simulink model "Lcontainer_simNN"  (R2018b)
settings: Solver=FixedStepAuto  StartTime=0.0  StopTime=50  FixedStep=0.1  RelTol=1e-3
libraries: neural x548, simulink x2
(part 10 of 26)

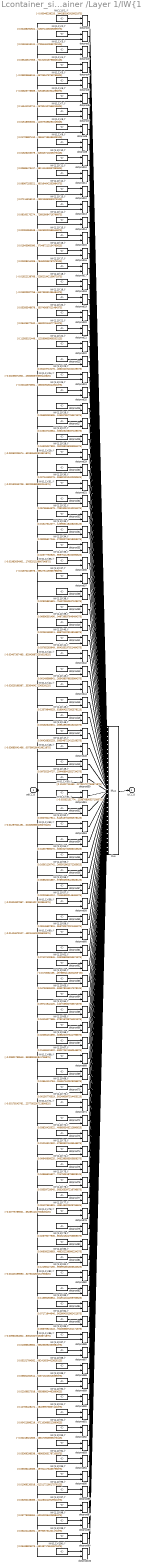
== system Lcontainer_simNN/Lcontainer Plant/NN Plant2 LContainer /Layer 1/IW{1,1} ==
  "pd{1,1}" : Inport  PortDimensions=10
      mask Display: e = 0.06;c1 = [120 230 180]/255;c2 = ([120 230 180]+0)/(256+128);c3 = ([120 230 180]+128)/(256+128);patch([0 1 1 0],[0 0 1 1],c1);patch([0 1 1 1-e 1-e 0+e],[0 0 1 1-e 0+e 0+e],c2);patch([0 0 1 1-e 0+e 0+e],[0 1 1 1-e 1-e 0+e],c3);plot([0 1 1 0 0],[0 0 1 1 0]);
  "IW{1,1}(1,:)'" : Constant  Value=[-0.0094623922020518891340401523848413489758968353271484375;-0.09558953457089498784160497280026902444660663604736328125;0.26068741035971088049194577251910232007503509521484375;-0.0982085917647781136974316495980019681155681610107421875;0.0376402374620294077889326445074402727186679840087890625;0.130169172499156327038605240886681713163852691650390625;0.09123082026825020396376686449002590961754322052001953125;0.08727806527434033012635694603886804543435573577880859375;0.06335140080853875199640157234171056188642978668212890625;-0.019497242791725710731043363921344280242919921875]
      mask Display: e = 0.06;c1 = [120 150 230]/255;c2 = ([120 150 230]+0)/383;c3 = ([120 150 230]+128)/383;patch([0 1 1 0],[0 0 1 1],c1);patch([0 1 1 1-e 1-e 0+e],[0 0 1 1-e 0+e 0+e],c2);patch([0 0 1 1-e 0+e 0+e],[0 1 1 1-e 1-e 0+e],c3);plot([0 1 1 0 0],[0 0 1 1 0]);disp('Weights');
  "IW{1,1}(10,:)'" : Constant  Value=[0.01626203379415903926830111458912142552435398101806640625;-0.0116878579195638099275100785234826616942882537841796875;0.1330582734436684677614692873248714022338390350341796875;0.0022158363261503325435108902041747569455765187740325927734375;-0.054351051398197784692012390905802021734416484832763671875;-0.132257520166433051311827284735045395791530609130859375;0.06380697006039735830196235610856092534959316253662109375;0.249931899969640769487710940666147507727146148681640625;0.1755681253698809507479694502762868069112300872802734375;-0.00686988456380069507922758731410795007832348346710205078125]
      mask Display: e = 0.06;c1 = [120 150 230]/255;c2 = ([120 150 230]+0)/383;c3 = ([120 150 230]+128)/383;patch([0 1 1 0],[0 0 1 1],c1);patch([0 1 1 1-e 1-e 0+e],[0 0 1 1-e 0+e 0+e],c2);patch([0 0 1 1-e 0+e 0+e],[0 1 1 1-e 1-e 0+e],c3);plot([0 1 1 0 0],[0 0 1 1 0]);disp('Weights');
  "IW{1,1}(100,:)'" : Constant  Value=[0.05438825373927226591863615112742991186678409576416015625;-0.061530743551016668646536089681831072084605693817138671875;0.048468771448505997001543477153973071835935115814208984375;-0.01930008978486430493148873210884630680084228515625;-0.053213138463751592788231192798775737173855304718017578125;-0.1481686150629234755005114720916026271879673004150390625;-0.021741347273508182524892617948353290557861328125;0.059229112139614438492518644352458068169653415679931640625;-0.0278726089912357984090807150323598762042820453643798828125;-0.000331265188881957567228198069386735369334928691387176513671875]
      mask Display: e = 0.06;c1 = [120 150 230]/255;c2 = ([120 150 230]+0)/383;c3 = ([120 150 230]+128)/383;patch([0 1 1 0],[0 0 1 1],c1);patch([0 1 1 1-e 1-e 0+e],[0 0 1 1-e 0+e 0+e],c2);patch([0 0 1 1-e 0+e 0+e],[0 1 1 1-e 1-e 0+e],c3);plot([0 1 1 0 0],[0 0 1 1 0]);disp('Weights');
  "IW{1,1}(11,:)'" : Constant  Value=[0.00685473417855186374636478063848699093796312808990478515625;-0.07957314826937157692388069563094177283346652984619140625;0.0831181659954757512398515473250881768763065338134765625;-0.0018459122357845875010695646523117829929105937480926513671875;0.1496921802543421387010624812319292686879634857177734375;0.56792634713675183011361013996065594255924224853515625;0.044275812285080873298426240580738522112369537353515625;0.07070165839502252913550961466171429492533206939697265625;-0.1068912356905150906616341899280087091028690338134765625;0.0091264008795984043198590285328464233316481113433837890625]
      mask Display: e = 0.06;c1 = [120 150 230]/255;c2 = ([120 150 230]+0)/383;c3 = ([120 150 230]+128)/383;patch([0 1 1 0],[0 0 1 1],c1);patch([0 1 1 1-e 1-e 0+e],[0 0 1 1-e 0+e 0+e],c2);patch([0 0 1 1-e 0+e 0+e],[0 1 1 1-e 1-e 0+e],c3);plot([0 1 1 0 0],[0 0 1 1 0]);disp('Weights');
  "IW{1,1}(12,:)'" : Constant  Value=[0.089872555212271276747770798465353436768054962158203125;0.0085118080986059420356415472497246810235083103179931640625;-0.184376627901358058903014125462505035102367401123046875;0.0355803687804530088811816312954761087894439697265625;-0.005487872883921422577369053641405116650275886058807373046875;0.005156923061268266390844150492966946330852806568145751953125;0.11555051477834497875019081902792095206677913665771484375;-0.1686685266223485746284183051102445460855960845947265625;0.085807423146687877846261471859179437160491943359375;0.00411842000985169175153455256577217369340360164642333984375]
      mask Display: e = 0.06;c1 = [120 150 230]/255;c2 = ([120 150 230]+0)/383;c3 = ([120 150 230]+128)/383;patch([0 1 1 0],[0 0 1 1],c1);patch([0 1 1 1-e 1-e 0+e],[0 0 1 1-e 0+e 0+e],c2);patch([0 0 1 1-e 0+e 0+e],[0 1 1 1-e 1-e 0+e],c3);plot([0 1 1 0 0],[0 0 1 1 0]);disp('Weights');
  "IW{1,1}(13,:)'" : Constant  Value=[0.07114816112372672474162271782915922813117504119873046875;-0.032060096051675888995102781109380885027348995208740234375;0.0693593021014935195989181693221325986087322235107421875;0.034399420874747461962517292022312176413834095001220703125;0.02279928598992718435933824139283387921750545501708984375;-0.1450550631977100268787950199111946858465671539306640625;-0.08420904186461160290111394033374381251633167266845703125;0.25200435694978751133277228291262872517108917236328125;-0.060202799283688344933462843755478388629853725433349609375;0.032340333264820504688419333660931442864239215850830078125]
      mask Display: e = 0.06;c1 = [120 150 230]/255;c2 = ([120 150 230]+0)/383;c3 = ([120 150 230]+128)/383;patch([0 1 1 0],[0 0 1 1],c1);patch([0 1 1 1-e 1-e 0+e],[0 0 1 1-e 0+e 0+e],c2);patch([0 0 1 1-e 0+e 0+e],[0 1 1 1-e 1-e 0+e],c3);plot([0 1 1 0 0],[0 0 1 1 0]);disp('Weights');
  "IW{1,1}(14,:)'" : Constant  Value=[0.0816017027410976536483389054410508833825588226318359375;-0.0137702046599115536518187496994869434274733066558837890625;0.061825816425708612911193995387293398380279541015625;0.0182137031645154788550566848925882368348538875579833984375;0.016677444090910188700949134954498731531202793121337890625;-0.039017819642140079416936515599445556290447711944580078125;-0.0167140048186341406977195589433904387988150119781494140625;0.04790839033382394973603624066527117975056171417236328125;-0.08777787377106559263406637683146982453763484954833984375;0.01308305917827646928930374059518726426176726818084716796875]
      mask Display: e = 0.06;c1 = [120 150 230]/255;c2 = ([120 150 230]+0)/383;c3 = ([120 150 230]+128)/383;patch([0 1 1 0],[0 0 1 1],c1);patch([0 1 1 1-e 1-e 0+e],[0 0 1 1-e 0+e 0+e],c2);patch([0 0 1 1-e 0+e 0+e],[0 1 1 1-e 1-e 0+e],c3);plot([0 1 1 0 0],[0 0 1 1 0]);disp('Weights');
  "IW{1,1}(15,:)'" : Constant  Value=[0.0209195394819808623554369120256524183787405490875244140625;-0.009076813538002957704176054676281637512147426605224609375;0.1191679137212347805441226000766619108617305755615234375;0.002321578223835426245391655442062983638606965541839599609375;0.0685148415021334944441377956536598503589630126953125;-0.00157011605704497647119366465773282470763660967350006103515625;0.028108168660927877746669167891013785265386104583740234375;0.09391932602724477330280450360078248195350170135498046875;0.0284578772298975553323163723007382941432297229766845703125;0.005212281091639135548188033197902768733911216259002685546875]
      mask Display: e = 0.06;c1 = [120 150 230]/255;c2 = ([120 150 230]+0)/383;c3 = ([120 150 230]+128)/383;patch([0 1 1 0],[0 0 1 1],c1);patch([0 1 1 1-e 1-e 0+e],[0 0 1 1-e 0+e 0+e],c2);patch([0 0 1 1-e 0+e 0+e],[0 1 1 1-e 1-e 0+e],c3);plot([0 1 1 0 0],[0 0 1 1 0]);disp('Weights');
  "IW{1,1}(16,:)'" : Constant  Value=[0.0184396009007578264016213864806559286080300807952880859375;0.08622273237960843828009416256463737227022647857666015625;0.258984762037696547576359762388165108859539031982421875;0.007701939757252318670410762280198468943126499652862548828125;0.062159638552036954040058702730675577186048030853271484375;-0.11836257965172251871432962389008025638759136199951171875;0.0150200818445607904572103308282748912461102008819580078125;0.1617989899896752070684868840544368140399456024169921875;-0.0188621771444243309379107387258045491762459278106689453125;0.02152205623300353087845593336169258691370487213134765625]
      mask Display: e = 0.06;c1 = [120 150 230]/255;c2 = ([120 150 230]+0)/383;c3 = ([120 150 230]+128)/383;patch([0 1 1 0],[0 0 1 1],c1);patch([0 1 1 1-e 1-e 0+e],[0 0 1 1-e 0+e 0+e],c2);patch([0 0 1 1-e 0+e 0+e],[0 1 1 1-e 1-e 0+e],c3);plot([0 1 1 0 0],[0 0 1 1 0]);disp('Weights');
  "IW{1,1}(17,:)'" : Constant  Value=[0.0230831400684185332472520002511373604647815227508544921875;0.0667508846304031011609225743086426518857479095458984375;0.05900184207744356423841480818737181834876537322998046875;0.0167153228695464568798190185816565644927322864532470703125;-0.000672966141541886928890969787886433550738729536533355712890625;0.1782018798922027913445020885774283669888973236083984375;0.07145595567735839315215429223826504312455654144287109375;0.04002558594403750336088165795445092953741550445556640625;-0.1367353179557696252199860964537947438657283782958984375;0.004458470848905435497677718359454956953413784503936767578125]
      mask Display: e = 0.06;c1 = [120 150 230]/255;c2 = ([120 150 230]+0)/383;c3 = ([120 150 230]+128)/383;patch([0 1 1 0],[0 0 1 1],c1);patch([0 1 1 1-e 1-e 0+e],[0 0 1 1-e 0+e 0+e],c2);patch([0 0 1 1-e 0+e 0+e],[0 1 1 1-e 1-e 0+e],c3);plot([0 1 1 0 0],[0 0 1 1 0]);disp('Weights');
  "IW{1,1}(18,:)'" : Constant  Value=[-0.0182213876655290263339992407054523937404155731201171875;-0.000399743420678597030475109885827578182215802371501922607421875;-0.050901316682216070363953264177325763739645481109619140625;0.0250893053095773109484323271090033813379704952239990234375;0.08090673602776325690211223218284430913627147674560546875;0.0938809802481468669288489081736770458519458770751953125;0.0198702950067176260795509534773373161442577838897705078125;-0.057703964383789975445271380749545642174780368804931640625;-0.04276041067470219558810384796743164770305156707763671875;0.01306358593354533907671122250349071691744029521942138671875]
      mask Display: e = 0.06;c1 = [120 150 230]/255;c2 = ([120 150 230]+0)/383;c3 = ([120 150 230]+128)/383;patch([0 1 1 0],[0 0 1 1],c1);patch([0 1 1 1-e 1-e 0+e],[0 0 1 1-e 0+e 0+e],c2);patch([0 0 1 1-e 0+e 0+e],[0 1 1 1-e 1-e 0+e],c3);plot([0 1 1 0 0],[0 0 1 1 0]);disp('Weights');
  "IW{1,1}(19,:)'" : Constant  Value=[-0.018209377569535119267829514910772559233009815216064453125;-0.016649902739864948231218733099012752063572406768798828125;-0.004527751093878955822302767586506888619624078273773193359375;-0.0068852252691341438162186960880717379041016101837158203125;0.02209772471243469371682266455536591820418834686279296875;0.046415344483233873795757773450532113201916217803955078125;-0.004664568795302062066687742714066189364530146121978759765625;-0.01713973095097658105867566291635739617049694061279296875;-0.01135203955323040893310437837726567522622644901275634765625;-0.008753261637478436385517710505155264399945735931396484375]
      mask Display: e = 0.06;c1 = [120 150 230]/255;c2 = ([120 150 230]+0)/383;c3 = ([120 150 230]+128)/383;patch([0 1 1 0],[0 0 1 1],c1);patch([0 1 1 1-e 1-e 0+e],[0 0 1 1-e 0+e 0+e],c2);patch([0 0 1 1-e 0+e 0+e],[0 1 1 1-e 1-e 0+e],c3);plot([0 1 1 0 0],[0 0 1 1 0]);disp('Weights');
  "IW{1,1}(2,:)'" : Constant  Value=[0.004882929243012936425250014593757441616617143154144287109375;-0.057596398999574770216636210307115106843411922454833984375;-0.044082564852459558968345021412460482679307460784912109375;-0.01406400921559781795611154819880539434961974620819091796875;-0.0207834799436826568597158626516829826869070529937744140625;-0.12500641299832937480829286869266070425510406494140625;0.010192874151138286986650882681715302169322967529296875;0.08502904507598389727274224014763603918254375457763671875;0.141777425947241242365493008037446998059749603271484375;0.002150746476123398774615846917868111631833016872406005859375]
      mask Display: e = 0.06;c1 = [120 150 230]/255;c2 = ([120 150 230]+0)/383;c3 = ([120 150 230]+128)/383;patch([0 1 1 0],[0 0 1 1],c1);patch([0 1 1 1-e 1-e 0+e],[0 0 1 1-e 0+e 0+e],c2);patch([0 0 1 1-e 0+e 0+e],[0 1 1 1-e 1-e 0+e],c3);plot([0 1 1 0 0],[0 0 1 1 0]);disp('Weights');
  "IW{1,1}(20,:)'" : Constant  Value=[0.053935486796124150477016456761703011579811573028564453125;-0.0031300549363098115369929974605156530742533504962921142578125;0.09777932299305640284625695812792400829493999481201171875;-0.0341856829207596302211413785698823630809783935546875;0.1637615555876408279800671152770519256591796875;0.55379762131474119524199295483413152396678924560546875;0.049984170569442522291669916967293829657137393951416015625;-0.239524968831588969120360843589878641068935394287109375;0.1618070812272489888972160088087548501789569854736328125;0.027466021220655834067514433627366088330745697021484375]
      mask Display: e = 0.06;c1 = [120 150 230]/255;c2 = ([120 150 230]+0)/383;c3 = ([120 150 230]+128)/383;patch([0 1 1 0],[0 0 1 1],c1);patch([0 1 1 1-e 1-e 0+e],[0 0 1 1-e 0+e 0+e],c2);patch([0 0 1 1-e 0+e 0+e],[0 1 1 1-e 1-e 0+e],c3);plot([0 1 1 0 0],[0 0 1 1 0]);disp('Weights');
  "IW{1,1}(21,:)'" : Constant  Value=[0.054256779428249753138846500633007963187992572784423828125;-0.11238736437717598837249255439019179902970790863037109375;-0.1293053208545835996989836758075398392975330352783203125;0.0220913833444768455127604767085358616895973682403564453125;-0.03223635894362240905675065505420207045972347259521484375;0.10098705478395973711425170904476544819772243499755859375;-0.019627013149193052454766217351789237000048160552978515625;0.061199006731056944385915841166934114880859851837158203125;0.084865917404867874385132608949788846075534820556640625;0.04309910366681900251162318227216019295156002044677734375]
      mask Display: e = 0.06;c1 = [120 150 230]/255;c2 = ([120 150 230]+0)/383;c3 = ([120 150 230]+128)/383;patch([0 1 1 0],[0 0 1 1],c1);patch([0 1 1 1-e 1-e 0+e],[0 0 1 1-e 0+e 0+e],c2);patch([0 0 1 1-e 0+e 0+e],[0 1 1 1-e 1-e 0+e],c3);plot([0 1 1 0 0],[0 0 1 1 0]);disp('Weights');
  "IW{1,1}(22,:)'" : Constant  Value=[0.1158315144990087475207474199123680591583251953125;-0.1634728196516810616589765459139016456902027130126953125;0.035020493849886764892165302853754837997257709503173828125;0.0111778835228135246804281877075482043437659740447998046875;-0.0561490815014391575488161834073252975940704345703125;-0.2146205341687602297096049142055562697350978851318359375;0.11055470925725384423454755733473575673997402191162109375;0.0154180878450160437076466024564069812186062335968017578125;0.066143219849594092618616514300811104476451873779296875;0.033149436754358004020293293478971463628113269805908203125]
      mask Display: e = 0.06;c1 = [120 150 230]/255;c2 = ([120 150 230]+0)/383;c3 = ([120 150 230]+128)/383;patch([0 1 1 0],[0 0 1 1],c1);patch([0 1 1 1-e 1-e 0+e],[0 0 1 1-e 0+e 0+e],c2);patch([0 0 1 1-e 0+e 0+e],[0 1 1 1-e 1-e 0+e],c3);plot([0 1 1 0 0],[0 0 1 1 0]);disp('Weights');
  "IW{1,1}(23,:)'" : Constant  Value=[0.00419713176387549909140961545972459134645760059356689453125;0.1170293572207423693498640204779803752899169921875;0.05992652827845613983104300359627814032137393951416015625;0.0027034221247037859559014805199694819748401641845703125;-0.0184799404250086708734190921177287236787378787994384765625;0.1485927881894391067163496700231917202472686767578125;-0.053373316924542467398762113361954106949269771575927734375;-0.041164967862770511508596626981670851819217205047607421875;0.0661805237237923782434023678433732129633426666259765625;0.00348532813765325098775971213171942508779466152191162109375]
      mask Display: e = 0.06;c1 = [120 150 230]/255;c2 = ([120 150 230]+0)/383;c3 = ([120 150 230]+128)/383;patch([0 1 1 0],[0 0 1 1],c1);patch([0 1 1 1-e 1-e 0+e],[0 0 1 1-e 0+e 0+e],c2);patch([0 0 1 1-e 0+e 0+e],[0 1 1 1-e 1-e 0+e],c3);plot([0 1 1 0 0],[0 0 1 1 0]);disp('Weights');
  "IW{1,1}(24,:)'" : Constant  Value=[-0.0023667490167734671867305618064847294590435922145843505859375;-0.0026621574457762827055351539939920257893390953540802001953125;0.098039684675983007622335207997821271419525146484375;0.0219371829502120647970020428374482435174286365509033203125;-0.02163029214711008341165410229223198257386684417724609375;0.1095352711170798354345379266305826604366302490234375;-0.01500366036165250681333471760581232956610620021820068359375;0.04497043112273464704475856024146196432411670684814453125;-0.025171986185772356192646981298821629025042057037353515625;0.01015432471195599518909435943214703002013266086578369140625]
      mask Display: e = 0.06;c1 = [120 150 230]/255;c2 = ([120 150 230]+0)/383;c3 = ([120 150 230]+128)/383;patch([0 1 1 0],[0 0 1 1],c1);patch([0 1 1 1-e 1-e 0+e],[0 0 1 1-e 0+e 0+e],c2);patch([0 0 1 1-e 0+e 0+e],[0 1 1 1-e 1-e 0+e],c3);plot([0 1 1 0 0],[0 0 1 1 0]);disp('Weights');
  "IW{1,1}(25,:)'" : Constant  Value=[-0.000428708940112308288690468049964010788244195282459259033203125;9.1544086241367931926216083837744008633308112621307373046875e-05;-0.0004300533793372667413883181364298025073367170989513397216796875;6.48029488285427335281241312259226106107234954833984375e-05;-0.00129145474964229727866948937986535383970476686954498291015625;-0.0020837039570330271633091800964621143066324293613433837890625;-0.0004094497946522885679400405312122757095494307577610015869140625;0.0001162733233937415983950958153769761338480748236179351806640625;-0.00016801208466965373796754568136435636915848590433597564697265625;-0.0002100271527808877133729204000900381288374774158000946044921875]
      mask Display: e = 0.06;c1 = [120 150 230]/255;c2 = ([120 150 230]+0)/383;c3 = ([120 150 230]+128)/383;patch([0 1 1 0],[0 0 1 1],c1);patch([0 1 1 1-e 1-e 0+e],[0 0 1 1-e 0+e 0+e],c2);patch([0 0 1 1-e 0+e 0+e],[0 1 1 1-e 1-e 0+e],c3);plot([0 1 1 0 0],[0 0 1 1 0]);disp('Weights');
  "IW{1,1}(26,:)'" : Constant  Value=[0.055892806950742328353509691396538983099162578582763671875;-0.1284268204621448195013044824008829891681671142578125;-0.0635938515163453066403320690369582735002040863037109375;0.0278544960430266476392180408083731890656054019927978515625;0.0018930102148548813741080198980171189759857952594757080078125;-0.090385076943400533000527730109752155840396881103515625;0.132461038461452684789065870063495822250843048095703125;0.13139818141287362696090212921262718737125396728515625;0.1367989270820009484186385861903545446693897247314453125;-0.0002401367004118174180819778040785195116768591105937957763671875]
      mask Display: e = 0.06;c1 = [120 150 230]/255;c2 = ([120 150 230]+0)/383;c3 = ([120 150 230]+128)/383;patch([0 1 1 0],[0 0 1 1],c1);patch([0 1 1 1-e 1-e 0+e],[0 0 1 1-e 0+e 0+e],c2);patch([0 0 1 1-e 0+e 0+e],[0 1 1 1-e 1-e 0+e],c3);plot([0 1 1 0 0],[0 0 1 1 0]);disp('Weights');
  "IW{1,1}(27,:)'" : Constant  Value=[0.1061671838416390067916239559053792618215084075927734375;0.01455106568329974682518557216326371417380869388580322265625;0.2194665097169405110211215514937066473066806793212890625;0.01436225965540223643845951784214776125736534595489501953125;-0.0997290353010053809423851589599507860839366912841796875;-0.51024718783592548643213149262010119855403900146484375;-7.5215616431395691744883624796358390085515566170215606689453125e-05;0.046546095145313791385799362387842847965657711029052734375;-0.054755540426459102520961863547199754975736141204833984375;-0.01035067696942139868487853249234831309877336025238037109375]
      mask Display: e = 0.06;c1 = [120 150 230]/255;c2 = ([120 150 230]+0)/383;c3 = ([120 150 230]+128)/383;patch([0 1 1 0],[0 0 1 1],c1);patch([0 1 1 1-e 1-e 0+e],[0 0 1 1-e 0+e 0+e],c2);patch([0 0 1 1-e 0+e 0+e],[0 1 1 1-e 1-e 0+e],c3);plot([0 1 1 0 0],[0 0 1 1 0]);disp('Weights');
  "IW{1,1}(28,:)'" : Constant  Value=[0.043250379936406797842796123632069793529808521270751953125;0.049753204596124860070727180527683231048285961151123046875;-0.1329378169960137856531190436726319603621959686279296875;0.01885286933153483557301655082483193837106227874755859375;0.046117914719532533684986930211380240507423877716064453125;0.35414050109305106328605461385450325906276702880859375;-0.033653993165451250024755580625424045138061046600341796875;-0.003085228111936642002299802101106251939199864864349365234375;-0.07851150253082912755520084147065063007175922393798828125;0.036814308916874725896573039563008933328092098236083984375]
      mask Display: e = 0.06;c1 = [120 150 230]/255;c2 = ([120 150 230]+0)/383;c3 = ([120 150 230]+128)/383;patch([0 1 1 0],[0 0 1 1],c1);patch([0 1 1 1-e 1-e 0+e],[0 0 1 1-e 0+e 0+e],c2);patch([0 0 1 1-e 0+e 0+e],[0 1 1 1-e 1-e 0+e],c3);plot([0 1 1 0 0],[0 0 1 1 0]);disp('Weights');
  "IW{1,1}(29,:)'" : Constant  Value=[-0.030620255742750242256011716790453647263348102569580078125;-0.060072751731736630242952656999477767385542392730712890625;0.035252039674856010254000437953436630778014659881591796875;-0.00919170816308433925867493741179714561440050601959228515625;0.023535161861715871156608415049049654044210910797119140625;0.2258211689467672644848761365210521034896373748779296875;-0.00230639337737633016989224898907195893116295337677001953125;0.007157763388058989602324988510417824727483093738555908203125;-0.1325624286244390936939652192450012080371379852294921875;-0.00019654571167457865303596076245185031439177691936492919921875]
      mask Display: e = 0.06;c1 = [120 150 230]/255;c2 = ([120 150 230]+0)/383;c3 = ([120 150 230]+128)/383;patch([0 1 1 0],[0 0 1 1],c1);patch([0 1 1 1-e 1-e 0+e],[0 0 1 1-e 0+e 0+e],c2);patch([0 0 1 1-e 0+e 0+e],[0 1 1 1-e 1-e 0+e],c3);plot([0 1 1 0 0],[0 0 1 1 0]);disp('Weights');
  "IW{1,1}(3,:)'" : Constant  Value=[0.01504613241257331084088644246321564423851668834686279296875;-0.018507599401025205676507567886801552958786487579345703125;0.0418247693695602273944444959852262400090694427490234375;-0.09051438570647639403343731601125909946858882904052734375;-0.0171372621545999026526629904765286482870578765869140625;-0.170833727731954432282890365968341939151287078857421875;-0.0035696038583175608745190476867037432384677231311798095703125;-0.034239869832726803344780108773193205706775188446044921875;0.0251699400853839481972951119814752019010484218597412109375;-0.000573952465504741493607099300788831897079944610595703125]
      mask Display: e = 0.06;c1 = [120 150 230]/255;c2 = ([120 150 230]+0)/383;c3 = ([120 150 230]+128)/383;patch([0 1 1 0],[0 0 1 1],c1);patch([0 1 1 1-e 1-e 0+e],[0 0 1 1-e 0+e 0+e],c2);patch([0 0 1 1-e 0+e 0+e],[0 1 1 1-e 1-e 0+e],c3);plot([0 1 1 0 0],[0 0 1 1 0]);disp('Weights');
  "IW{1,1}(30,:)'" : Constant  Value=[0.027341892766545104753728168134330189786851406097412109375;0.1252022346316188639026023565747891552746295928955078125;-0.0110998452900594561654212810708486358635127544403076171875;0.049645084866596599082466667596236220560967922210693359375;-0.04948149832591917929303093615089892409741878509521484375;-0.059672753066025006896122562238815589807927608489990234375;0.021246913175135127838100146391298039816319942474365234375;0.10083037720781040658124538822448812425136566162109375;0.0601722007103199507671575929634855128824710845947265625;0.005628721429224396201329572164695491665042936801910400390625]
      mask Display: e = 0.06;c1 = [120 150 230]/255;c2 = ([120 150 230]+0)/383;c3 = ([120 150 230]+128)/383;patch([0 1 1 0],[0 0 1 1],c1);patch([0 1 1 1-e 1-e 0+e],[0 0 1 1-e 0+e 0+e],c2);patch([0 0 1 1-e 0+e 0+e],[0 1 1 1-e 1-e 0+e],c3);plot([0 1 1 0 0],[0 0 1 1 0]);disp('Weights');
  "IW{1,1}(31,:)'" : Constant  Value=[-0.001300457083481666546720401100856179255060851573944091796875;0.0029817332399571555741346617907083782483823597431182861328125;-0.0035784949147766999082154182332260461407713592052459716796875;0.004177790401596108600668078025819340837188065052032470703125;-0.01019553427399688162735547081183540285564959049224853515625;-0.0160996964297110585484507083720018272288143634796142578125;-0.002441254860139726277912242125012198812328279018402099609375;0.0031805179703750029000797194811411827686242759227752685546875;-0.000631347408235451829604245599369960473268292844295501708984375;-0.000638603839496102907401231529860297086997888982295989990234375]
      mask Display: e = 0.06;c1 = [120 150 230]/255;c2 = ([120 150 230]+0)/383;c3 = ([120 150 230]+128)/383;patch([0 1 1 0],[0 0 1 1],c1);patch([0 1 1 1-e 1-e 0+e],[0 0 1 1-e 0+e 0+e],c2);patch([0 0 1 1-e 0+e 0+e],[0 1 1 1-e 1-e 0+e],c3);plot([0 1 1 0 0],[0 0 1 1 0]);disp('Weights');
  "IW{1,1}(32,:)'" : Constant  Value=[0.057655645798538823765255756370606832206249237060546875;0.0175213535064214949443783808646912802942097187042236328125;0.167545314656773414174750769234378822147846221923828125;0.01435359908537950542062322512038008426316082477569580078125;-0.0424012483635934633863229237249470315873622894287109375;-0.1755816998638709824920312030371860601007938385009765625;-0.026032023806178118674470312043922604061663150787353515625;0.1070502049234766384078199052964919246733188629150390625;-0.04798256895018682133269294354249723255634307861328125;0.023793277194497496063174679648000164888799190521240234375]
      mask Display: e = 0.06;c1 = [120 150 230]/255;c2 = ([120 150 230]+0)/383;c3 = ([120 150 230]+128)/383;patch([0 1 1 0],[0 0 1 1],c1);patch([0 1 1 1-e 1-e 0+e],[0 0 1 1-e 0+e 0+e],c2);patch([0 0 1 1-e 0+e 0+e],[0 1 1 1-e 1-e 0+e],c3);plot([0 1 1 0 0],[0 0 1 1 0]);disp('Weights');
  "IW{1,1}(33,:)'" : Constant  Value=[0.0154751207722963191049103670593467541038990020751953125;-0.06508292427735633267626980114073376171290874481201171875;0.003597379266779768790252003185514695360325276851654052734375;-0.01217999549635321275553589970286338939331471920013427734375;-0.024807022455973541663620807184997829608619213104248046875;0.245955434496933078580838127891183830797672271728515625;0.054715556931545165919583695313122007064521312713623046875;0.00124258971353589388851579311534578664577566087245941162109375;0.044862425392990117056779553195156040601432323455810546875;0.0021306295208748525678299490238032376510091125965118408203125]
      mask Display: e = 0.06;c1 = [120 150 230]/255;c2 = ([120 150 230]+0)/383;c3 = ([120 150 230]+128)/383;patch([0 1 1 0],[0 0 1 1],c1);patch([0 1 1 1-e 1-e 0+e],[0 0 1 1-e 0+e 0+e],c2);patch([0 0 1 1-e 0+e 0+e],[0 1 1 1-e 1-e 0+e],c3);plot([0 1 1 0 0],[0 0 1 1 0]);disp('Weights');
  "IW{1,1}(34,:)'" : Constant  Value=[0.0829561724641332265406390433781780302524566650390625;-0.08643372278495968508149616127411718480288982391357421875;0.02650072339475682825504776474190293811261653900146484375;-0.010102262395204252010127987659870996139943599700927734375;-0.0170359998743756478611910409881602390669286251068115234375;-0.2137723706639365894854876160025014542043209075927734375;0.1662215532799683204157048521665274165570735931396484375;0.1793015865651973184125012039658031426370143890380859375;0.044423895055723854052853738494377466849982738494873046875;0.006377591494637540291134936154548995546065270900726318359375]
      mask Display: e = 0.06;c1 = [120 150 230]/255;c2 = ([120 150 230]+0)/383;c3 = ([120 150 230]+128)/383;patch([0 1 1 0],[0 0 1 1],c1);patch([0 1 1 1-e 1-e 0+e],[0 0 1 1-e 0+e 0+e],c2);patch([0 0 1 1-e 0+e 0+e],[0 1 1 1-e 1-e 0+e],c3);plot([0 1 1 0 0],[0 0 1 1 0]);disp('Weights');
  "IW{1,1}(35,:)'" : Constant  Value=[0.0257775092536612245031069079459484783001244068145751953125;0.01013277491170373571793827949250044184736907482147216796875;0.1824594839372037646807456212627585045993328094482421875;-0.037732190422867024903741395291945082135498523712158203125;0.116527238491814066900786883707041852176189422607421875;0.446641372272815695421144255305989645421504974365234375;0.051285192038531483837981994611254776827991008758544921875;-0.049995574103856306458215641441711341030895709991455078125;-0.023550005796922769685242116111112409271299839019775390625;0.03835423208526923810612885290538542903959751129150390625]
      mask Display: e = 0.06;c1 = [120 150 230]/255;c2 = ([120 150 230]+0)/383;c3 = ([120 150 230]+128)/383;patch([0 1 1 0],[0 0 1 1],c1);patch([0 1 1 1-e 1-e 0+e],[0 0 1 1-e 0+e 0+e],c2);patch([0 0 1 1-e 0+e 0+e],[0 1 1 1-e 1-e 0+e],c3);plot([0 1 1 0 0],[0 0 1 1 0]);disp('Weights');
  "IW{1,1}(36,:)'" : Constant  Value=[-0.01983054901434673500393301992517081089317798614501953125;0.018452101329059479584149272568538435734808444976806640625;0.0032003306650281028271354255565483981627039611339569091796875;0.0189674161409785456411380977215230814181268215179443359375;-0.045544104438170647519701361716215615160763263702392578125;0.11854060794901606634699220421680365689098834991455078125;-0.03286269016840230594578287082185852341353893280029296875;0.2297929534733335332763459746274747885763645172119140625;0.2591117873913864055879230363643728196620941162109375;-0.0021468140763482713821719283231459485250525176525115966796875]
      mask Display: e = 0.06;c1 = [120 150 230]/255;c2 = ([120 150 230]+0)/383;c3 = ([120 150 230]+128)/383;patch([0 1 1 0],[0 0 1 1],c1);patch([0 1 1 1-e 1-e 0+e],[0 0 1 1-e 0+e 0+e],c2);patch([0 0 1 1-e 0+e 0+e],[0 1 1 1-e 1-e 0+e],c3);plot([0 1 1 0 0],[0 0 1 1 0]);disp('Weights');
  "IW{1,1}(37,:)'" : Constant  Value=[-0.01870216976054601965007151420650188811123371124267578125;-0.1487696091116151586586369148790254257619380950927734375;-0.042997654762433688835354672619359917007386684417724609375;-0.0157909863387145910085251898635760881006717681884765625;0.060172801600213599027000554997357539832592010498046875;0.295341177415798628036469608559855259954929351806640625;0.04437611723870467372865533661752124316990375518798828125;0.057450552118198931761394732120606931857764720916748046875;0.1758418061116827912915283604888827539980411529541015625;0.01235623289356558955620624118409978109411895275115966796875]
      mask Display: e = 0.06;c1 = [120 150 230]/255;c2 = ([120 150 230]+0)/383;c3 = ([120 150 230]+128)/383;patch([0 1 1 0],[0 0 1 1],c1);patch([0 1 1 1-e 1-e 0+e],[0 0 1 1-e 0+e 0+e],c2);patch([0 0 1 1-e 0+e 0+e],[0 1 1 1-e 1-e 0+e],c3);plot([0 1 1 0 0],[0 0 1 1 0]);disp('Weights');
  "IW{1,1}(38,:)'" : Constant  Value=[0.02925881681080506890868520031290245242416858673095703125;0.091494353634817338072338088750257156789302825927734375;-0.0067900404159471593190655624994178651832044124603271484375;0.006873783434484160952127052013338470715098083019256591796875;0.010202439038604564636170124458658392541110515594482421875;-0.0069640709699677165456233041140876593999564647674560546875;0.04781638241289569435377160289135645143687725067138671875;-0.041503627391795409884434064906599815003573894500732421875;-0.047215748285432075637135795886933919973671436309814453125;-0.000644734460318443516023412254156710332608781754970550537109375]
      mask Display: e = 0.06;c1 = [120 150 230]/255;c2 = ([120 150 230]+0)/383;c3 = ([120 150 230]+128)/383;patch([0 1 1 0],[0 0 1 1],c1);patch([0 1 1 1-e 1-e 0+e],[0 0 1 1-e 0+e 0+e],c2);patch([0 0 1 1-e 0+e 0+e],[0 1 1 1-e 1-e 0+e],c3);plot([0 1 1 0 0],[0 0 1 1 0]);disp('Weights');
  "IW{1,1}(39,:)'" : Constant  Value=[0.06696391490814442015722107726105605252087116241455078125;0.043507059958706455204957563864809344522655010223388671875;0.0022627982478876872661499586314448606572113931179046630859375;0.00592600017327450136195299279506798484362661838531494140625;0.024770048623384478825304455540390335954725742340087890625;-0.2191043250452577861864256192347966134548187255859375;0.024279235658779714512878200594059308059513568878173828125;0.136827226052908812459207865686039440333843231201171875;0.12302496885916480717781951170763932168483734130859375;0.042787993807286893443997399799627601169049739837646484375]
      mask Display: e = 0.06;c1 = [120 150 230]/255;c2 = ([120 150 230]+0)/383;c3 = ([120 150 230]+128)/383;patch([0 1 1 0],[0 0 1 1],c1);patch([0 1 1 1-e 1-e 0+e],[0 0 1 1-e 0+e 0+e],c2);patch([0 0 1 1-e 0+e 0+e],[0 1 1 1-e 1-e 0+e],c3);plot([0 1 1 0 0],[0 0 1 1 0]);disp('Weights');
  "IW{1,1}(4,:)'" : Constant  Value=[0.036406173535373155536465361592490808106958866119384765625;0.0303225872789273688534539274996859603561460971832275390625;0.016992587776736754745510182829093537293374538421630859375;0.0712699496276618382761824932458694092929363250732421875;-0.0922836711084928651427361501191626302897930145263671875;-0.0293263071250228178621366481593213393352925777435302734375;0.003353206534465286332846734040913361241109669208526611328125;0.003514382330419968218648829605399441788904368877410888671875;-0.07268810781557318023704539200480212457478046417236328125;-0.0020694202711757825503824381740969329257495701313018798828125]
      mask Display: e = 0.06;c1 = [120 150 230]/255;c2 = ([120 150 230]+0)/383;c3 = ([120 150 230]+128)/383;patch([0 1 1 0],[0 0 1 1],c1);patch([0 1 1 1-e 1-e 0+e],[0 0 1 1-e 0+e 0+e],c2);patch([0 0 1 1-e 0+e 0+e],[0 1 1 1-e 1-e 0+e],c3);plot([0 1 1 0 0],[0 0 1 1 0]);disp('Weights');
  "IW{1,1}(40,:)'" : Constant  Value=[0.0226246931135768401810448580135926022194325923919677734375;0.0609845520991494083329342856814037077128887176513671875;0.11617872595918903033673785785140353254973888397216796875;-0.0114620108114807418842051589535913080908358097076416015625;0.08985106470019448010599916187857161276042461395263671875;0.423456091179193749862719187149195931851863861083984375;-0.0841011889559413472472471084984135814011096954345703125;-0.032343871456650685747291618099552579224109649658203125;0.0187508808586528304129803501609785598702728748321533203125;0.053166644332708561104805511376980575732886791229248046875]
      mask Display: e = 0.06;c1 = [120 150 230]/255;c2 = ([120 150 230]+0)/383;c3 = ([120 150 230]+128)/383;patch([0 1 1 0],[0 0 1 1],c1);patch([0 1 1 1-e 1-e 0+e],[0 0 1 1-e 0+e 0+e],c2);patch([0 0 1 1-e 0+e 0+e],[0 1 1 1-e 1-e 0+e],c3);plot([0 1 1 0 0],[0 0 1 1 0]);disp('Weights');
  "IW{1,1}(41,:)'" : Constant  Value=[0.037652839492859212222608533693346544168889522552490234375;0.0706526518036562911628806205044384114444255828857421875;0.11989744985270396615550936303407070226967334747314453125;0.00365966674761863085263424721915725967846810817718505859375;0.017277339343304609631246648859814740717411041259765625;0.135125244957386814181887757513322867453098297119140625;0.00192273184513320843057326836600395836285315454006195068359375;-0.03252992580396761590488807769361301325261592864990234375;-0.102432590640903875556233515453641302883625030517578125;0.0065013752071739171201070206507210968993604183197021484375]
      mask Display: e = 0.06;c1 = [120 150 230]/255;c2 = ([120 150 230]+0)/383;c3 = ([120 150 230]+128)/383;patch([0 1 1 0],[0 0 1 1],c1);patch([0 1 1 1-e 1-e 0+e],[0 0 1 1-e 0+e 0+e],c2);patch([0 0 1 1-e 0+e 0+e],[0 1 1 1-e 1-e 0+e],c3);plot([0 1 1 0 0],[0 0 1 1 0]);disp('Weights');
  "IW{1,1}(42,:)'" : Constant  Value=[-0.034073074951517672015466331458810600452125072479248046875;0.0789402390914708818048239891140838153660297393798828125;0.0226947690121968824461529123936998075805604457855224609375;-0.0186643067981428732726723040968863642774522304534912109375;0.0280594575673095876500173773138158139772713184356689453125;0.27117506491122245204650198502349667251110076904296875;-0.054575703267962301368232402865032781846821308135986328125;0.0295706673640438420791465290449195890687406063079833984375;-0.1193862284205201851339239738081232644617557525634765625;-0.00906888053951409624231505546276821405626833438873291015625]
      mask Display: e = 0.06;c1 = [120 150 230]/255;c2 = ([120 150 230]+0)/383;c3 = ([120 150 230]+128)/383;patch([0 1 1 0],[0 0 1 1],c1);patch([0 1 1 1-e 1-e 0+e],[0 0 1 1-e 0+e 0+e],c2);patch([0 0 1 1-e 0+e 0+e],[0 1 1 1-e 1-e 0+e],c3);plot([0 1 1 0 0],[0 0 1 1 0]);disp('Weights');
  "IW{1,1}(43,:)'" : Constant  Value=[0.00149588641771458458369636890239462445606477558612823486328125;0.028824063696041679616399733276921324431896209716796875;0.034845924388722006315166623835466452874243259429931640625;-0.0272887302741802069416809928270595264621078968048095703125;0.05041316221349168014143060645437799394130706787109375;0.09148685717208689116564102050688234157860279083251953125;-0.10707755038642419176397879709838889539241790771484375;0.00887624718988880463677038079595149611122906208038330078125;-0.0960741601912546705488438192332978360354900360107421875;-0.0025010786829252340535134635501890443265438079833984375]
      mask Display: e = 0.06;c1 = [120 150 230]/255;c2 = ([120 150 230]+0)/383;c3 = ([120 150 230]+128)/383;patch([0 1 1 0],[0 0 1 1],c1);patch([0 1 1 1-e 1-e 0+e],[0 0 1 1-e 0+e 0+e],c2);patch([0 0 1 1-e 0+e 0+e],[0 1 1 1-e 1-e 0+e],c3);plot([0 1 1 0 0],[0 0 1 1 0]);disp('Weights');
  "IW{1,1}(44,:)'" : Constant  Value=[-0.0262919838708194873733159369066925137303769588470458984375;-0.09891711576821389517721883066769805736839771270751953125;0.171248082329450823646510571052203886210918426513671875;-0.031560906234920249602282638079486787319183349609375;0.0763710517151593715201585155227803625166416168212890625;0.84927724511108915184109946494572795927524566650390625;0.0881912324052968876753055837980355136096477508544921875;0.1364688751119919885024245331806014291942119598388671875;0.0151534903671480015996397838762277388013899326324462890625;0.00538303845850146740759090135952646960504353046417236328125]
      mask Display: e = 0.06;c1 = [120 150 230]/255;c2 = ([120 150 230]+0)/383;c3 = ([120 150 230]+128)/383;patch([0 1 1 0],[0 0 1 1],c1);patch([0 1 1 1-e 1-e 0+e],[0 0 1 1-e 0+e 0+e],c2);patch([0 0 1 1-e 0+e 0+e],[0 1 1 1-e 1-e 0+e],c3);plot([0 1 1 0 0],[0 0 1 1 0]);disp('Weights');
  "IW{1,1}(45,:)'" : Constant  Value=[0.13379846033323306020434984020539559423923492431640625;0.041478146715528636800929263017678749747574329376220703125;-0.08059196209386564058174684532787068746984004974365234375;0.03778851120177016686962900848811841569840908050537109375;-0.005282945967682390643604950497547179111279547214508056640625;-0.1279698649768603591070359470904804766178131103515625;-0.019188878855175194038107377991764224134385585784912109375;-0.01211062158931112790749562435621555778197944164276123046875;0.09436972662845211079485352456686086952686309814453125;0.03765781897895577323698290683751110918819904327392578125]
      mask Display: e = 0.06;c1 = [120 150 230]/255;c2 = ([120 150 230]+0)/383;c3 = ([120 150 230]+128)/383;patch([0 1 1 0],[0 0 1 1],c1);patch([0 1 1 1-e 1-e 0+e],[0 0 1 1-e 0+e 0+e],c2);patch([0 0 1 1-e 0+e 0+e],[0 1 1 1-e 1-e 0+e],c3);plot([0 1 1 0 0],[0 0 1 1 0]);disp('Weights');
  "IW{1,1}(46,:)'" : Constant  Value=[0.031826406319517393239681979366650921292603015899658203125;0.09134328812660989782568066175372223369777202606201171875;0.1876069824791513074302429231465794146060943603515625;-0.021759602034773894985164588433690369129180908203125;-0.1273349733162982833079013289534486830234527587890625;-0.2930394475669177989374247772502712905406951904296875;0.0190227768760909791978530591904927860014140605926513671875;0.01162750862308703676817334127235881169326603412628173828125;-0.019561777479921334255141829316926305182278156280517578125;0.006964629140588782761633890316943507059477269649505615234375]
      mask Display: e = 0.06;c1 = [120 150 230]/255;c2 = ([120 150 230]+0)/383;c3 = ([120 150 230]+128)/383;patch([0 1 1 0],[0 0 1 1],c1);patch([0 1 1 1-e 1-e 0+e],[0 0 1 1-e 0+e 0+e],c2);patch([0 0 1 1-e 0+e 0+e],[0 1 1 1-e 1-e 0+e],c3);plot([0 1 1 0 0],[0 0 1 1 0]);disp('Weights');
  "IW{1,1}(47,:)'" : Constant  Value=[0.0042683523343955143136696506189764477312564849853515625;-0.060383405865812790624946870821077027358114719390869140625;0.09097742607296969985508638956162030808627605438232421875;0.07017460644904345568040326952541363425552845001220703125;-0.12190030759358401468706034620481659658253192901611328125;0.1193899609977153997153465070368838496506214141845703125;-0.012087815457795525464490538070094771683216094970703125;0.23451678051623303655759400498936884105205535888671875;-0.11041275029647347472039342619609669782221317291259765625;-0.008752706717393497759527321022687829099595546722412109375]
      mask Display: e = 0.06;c1 = [120 150 230]/255;c2 = ([120 150 230]+0)/383;c3 = ([120 150 230]+128)/383;patch([0 1 1 0],[0 0 1 1],c1);patch([0 1 1 1-e 1-e 0+e],[0 0 1 1-e 0+e 0+e],c2);patch([0 0 1 1-e 0+e 0+e],[0 1 1 1-e 1-e 0+e],c3);plot([0 1 1 0 0],[0 0 1 1 0]);disp('Weights');
  "IW{1,1}(48,:)'" : Constant  Value=[-0.036850414661019785522722003179296734742820262908935546875;-0.0143346306495818580362122673932390171103179454803466796875;-0.12243746079234012202885395481644081883132457733154296875;-0.043567988709938713920433173143464955501258373260498046875;0.04097650099944903645532434666165499947965145111083984375;0.26224019627358075013034977018833160400390625;-0.0451321144566552978627527181743062101304531097412109375;0.015334501561122863833031004787699203006923198699951171875;0.0241995193336332244105069122497297939844429492950439453125;0.003314992381077605347605707919456108356826007366180419921875]
      mask Display: e = 0.06;c1 = [120 150 230]/255;c2 = ([120 150 230]+0)/383;c3 = ([120 150 230]+128)/383;patch([0 1 1 0],[0 0 1 1],c1);patch([0 1 1 1-e 1-e 0+e],[0 0 1 1-e 0+e 0+e],c2);patch([0 0 1 1-e 0+e 0+e],[0 1 1 1-e 1-e 0+e],c3);plot([0 1 1 0 0],[0 0 1 1 0]);disp('Weights');
  "IW{1,1}(49,:)'" : Constant  Value=[0.0975525473742113458097691136572393588721752166748046875;-0.055289432048035346001224610290591954253613948822021484375;0.029875013790731076712692271257765241898596286773681640625;0.021686151068051474910536313700504251755774021148681640625;0.046460429669174511946305727860817569307982921600341796875;-0.22034174891004043583819793639122508466243743896484375;-0.01089186020899320962718181959871799335815012454986572265625;0.0300068829149491185515064017863551271148025989532470703125;0.0306126046673695396960201975389281869865953922271728515625;0.01986654539378483741440817311740829609334468841552734375]
      mask Display: e = 0.06;c1 = [120 150 230]/255;c2 = ([120 150 230]+0)/383;c3 = ([120 150 230]+128)/383;patch([0 1 1 0],[0 0 1 1],c1);patch([0 1 1 1-e 1-e 0+e],[0 0 1 1-e 0+e 0+e],c2);patch([0 0 1 1-e 0+e 0+e],[0 1 1 1-e 1-e 0+e],c3);plot([0 1 1 0 0],[0 0 1 1 0]);disp('Weights');
  "IW{1,1}(5,:)'" : Constant  Value=[-0.0380366624494079264007240226419526152312755584716796875;-0.040528649545812485410767322946412605233490467071533203125;0.037328236215407088749440589481309871189296245574951171875;-0.0771374233431015576822886714580818079411983489990234375;-0.11020573303460590164348786856862716376781463623046875;-0.2614173502960517314619437456713058054447174072265625;0.053030182982346164843878710826174938119947910308837890625;0.0275453094931359006303228653678161208517849445343017578125;0.067418093142570689746406742415274493396282196044921875;-0.03503478743168264575302828234271146357059478759765625]
      mask Display: e = 0.06;c1 = [120 150 230]/255;c2 = ([120 150 230]+0)/383;c3 = ([120 150 230]+128)/383;patch([0 1 1 0],[0 0 1 1],c1);patch([0 1 1 1-e 1-e 0+e],[0 0 1 1-e 0+e 0+e],c2);patch([0 0 1 1-e 0+e 0+e],[0 1 1 1-e 1-e 0+e],c3);plot([0 1 1 0 0],[0 0 1 1 0]);disp('Weights');
  "IW{1,1}(50,:)'" : Constant  Value=[0.10422713463943873712924670371648971922695636749267578125;0.1083359301763390514228291294784867204725742340087890625;0.1461475110720540648845400255595450289547443389892578125;0.07898489549898625450286004934241645969450473785400390625;-0.10132036881906454628410330087717738933861255645751953125;-0.292117526291954809902762235651607625186443328857421875;0.1041519309197089793173063299036584794521331787109375;-0.01355163336700164998516182635057703009806573390960693359375;0.172598502126995401173559230301179923117160797119140625;0.01578803834081514423370862232332001440227031707763671875]
      mask Display: e = 0.06;c1 = [120 150 230]/255;c2 = ([120 150 230]+0)/383;c3 = ([120 150 230]+128)/383;patch([0 1 1 0],[0 0 1 1],c1);patch([0 1 1 1-e 1-e 0+e],[0 0 1 1-e 0+e 0+e],c2);patch([0 0 1 1-e 0+e 0+e],[0 1 1 1-e 1-e 0+e],c3);plot([0 1 1 0 0],[0 0 1 1 0]);disp('Weights');
  "IW{1,1}(51,:)'" : Constant  Value=[-0.0033313177466403249595006119676554590114392340183258056640625;-0.0341588628693798579405438431422226130962371826171875;-0.042509398866449298048930671711786999367177486419677734375;0.00843225605416361538579916867774954880587756633758544921875;0.023284114170592846992935420757930842228233814239501953125;0.13840070599917930760369699783041141927242279052734375;0.09118734390434686531978769608031143434345722198486328125;-0.0465043861848138673220631744698039256036281585693359375;0.07255082300809966022736574586815549992024898529052734375;0.0202320332612315433029603894965475774370133876800537109375]
      mask Display: e = 0.06;c1 = [120 150 230]/255;c2 = ([120 150 230]+0)/383;c3 = ([120 150 230]+128)/383;patch([0 1 1 0],[0 0 1 1],c1);patch([0 1 1 1-e 1-e 0+e],[0 0 1 1-e 0+e 0+e],c2);patch([0 0 1 1-e 0+e 0+e],[0 1 1 1-e 1-e 0+e],c3);plot([0 1 1 0 0],[0 0 1 1 0]);disp('Weights');
  "IW{1,1}(52,:)'" : Constant  Value=[0.00078247911638384634071263779020455331192351877689361572265625;0.00160347744452357080131854605298258320544846355915069580078125;-0.0033031084825199470873802187753653925028629601001739501953125;-0.06839373027485980138795440552712534554302692413330078125;-0.0157013038816831047850275382415929925628006458282470703125;-0.0412039339692927553127077544559142552316188812255859375;0.035196924275016062966248142629410722292959690093994140625;-0.0858582247768746864569067156480741687119007110595703125;0.0025895006501960881641066780645132894278503954410552978515625;-0.0064585838012340586467008307636206154711544513702392578125]
      mask Display: e = 0.06;c1 = [120 150 230]/255;c2 = ([120 150 230]+0)/383;c3 = ([120 150 230]+128)/383;patch([0 1 1 0],[0 0 1 1],c1);patch([0 1 1 1-e 1-e 0+e],[0 0 1 1-e 0+e 0+e],c2);patch([0 0 1 1-e 0+e 0+e],[0 1 1 1-e 1-e 0+e],c3);plot([0 1 1 0 0],[0 0 1 1 0]);disp('Weights');
  "IW{1,1}(53,:)'" : Constant  Value=[-0.0129762149148694161393535750903538428246974945068359375;0.140390383469986890219161068671382963657379150390625;0.00013868838886167832885089323813332384816021658480167388916015625;0.007069549182159425189386769972088586655445396900177001953125;-0.004966962334496720365972777244678582064807415008544921875;0.06995604035686701915874863288991036824882030487060546875;0.054296404826357162753946994371290202252566814422607421875;0.03617269796360710054639042709823115728795528411865234375;0.05815582579756418957206420827787951566278934478759765625;0.01292986339782160876143990435593877919018268585205078125]
      mask Display: e = 0.06;c1 = [120 150 230]/255;c2 = ([120 150 230]+0)/383;c3 = ([120 150 230]+128)/383;patch([0 1 1 0],[0 0 1 1],c1);patch([0 1 1 1-e 1-e 0+e],[0 0 1 1-e 0+e 0+e],c2);patch([0 0 1 1-e 0+e 0+e],[0 1 1 1-e 1-e 0+e],c3);plot([0 1 1 0 0],[0 0 1 1 0]);disp('Weights');
  "IW{1,1}(54,:)'" : Constant  Value=[0.043379892700374227121340453550146776251494884490966796875;0.055844174826941019029735713274931185878813266754150390625;0.036790948903711102879743322091599111445248126983642578125;0.002614072066953235760899953987745902850292623043060302734375;0.0291449259042995505175621673288333113305270671844482421875;-0.055446869668177183043678013518729130737483501434326171875;0.0152281209488946966956746109644882380962371826171875;0.0221353614566066787816556171719639678485691547393798828125;-0.09549934965343231940693158321664668619632720947265625;-0.0025116300600872437133459502689447617740370333194732666015625]
      mask Display: e = 0.06;c1 = [120 150 230]/255;c2 = ([120 150 230]+0)/383;c3 = ([120 150 230]+128)/383;patch([0 1 1 0],[0 0 1 1],c1);patch([0 1 1 1-e 1-e 0+e],[0 0 1 1-e 0+e 0+e],c2);patch([0 0 1 1-e 0+e 0+e],[0 1 1 1-e 1-e 0+e],c3);plot([0 1 1 0 0],[0 0 1 1 0]);disp('Weights');
  "IW{1,1}(55,:)'" : Constant  Value=[0.1656113074244591754080602186149917542934417724609375;0.0776434336671886493608241153197013773024082183837890625;0.006650712125608991553971094390362850390374660491943359375;0.053609677888561600711536669905399321578443050384521484375;-0.023284813740648890867390718995011411607265472412109375;-0.2747278714978824698533799164579249918460845947265625;0.09567299453889134552841966296909959055483341217041015625;-0.0614016000680394913313620008921134285628795623779296875;0.00012642444403650277885177433123686796534457243978977203369140625;0.0459189419882219118651534017772064544260501861572265625]
      mask Display: e = 0.06;c1 = [120 150 230]/255;c2 = ([120 150 230]+0)/383;c3 = ([120 150 230]+128)/383;patch([0 1 1 0],[0 0 1 1],c1);patch([0 1 1 1-e 1-e 0+e],[0 0 1 1-e 0+e 0+e],c2);patch([0 0 1 1-e 0+e 0+e],[0 1 1 1-e 1-e 0+e],c3);plot([0 1 1 0 0],[0 0 1 1 0]);disp('Weights');
  "IW{1,1}(56,:)'" : Constant  Value=[0.00862001887116782376796475517721773940138518810272216796875;0.04692958985582872111219643329604878090322017669677734375;0.0637131848196527406091860257220105268061161041259765625;-0.081765202577483819812442789043416269123554229736328125;0.107192047713503602057727448482182808220386505126953125;0.4226884419831347106111252287519164383411407470703125;0.09445914583771351791252612883909023366868495941162109375;0.150522884343338214652163742357515729963779449462890625;-0.08521705260338223453242534333185176365077495574951171875;0.000388683691411985843440490828726296967943198978900909423828125]
      mask Display: e = 0.06;c1 = [120 150 230]/255;c2 = ([120 150 230]+0)/383;c3 = ([120 150 230]+128)/383;patch([0 1 1 0],[0 0 1 1],c1);patch([0 1 1 1-e 1-e 0+e],[0 0 1 1-e 0+e 0+e],c2);patch([0 0 1 1-e 0+e 0+e],[0 1 1 1-e 1-e 0+e],c3);plot([0 1 1 0 0],[0 0 1 1 0]);disp('Weights');
  "IW{1,1}(57,:)'" : Constant  Value=[0.020266342122286763738348014385337592102587223052978515625;-0.049419302413537834206547216808758093975484371185302734375;0.126245260978732398715607132544391788542270660400390625;0.03484365749707414583458131573934224434196949005126953125;0.11833927247408020100305492405823315493762493133544921875;0.282917922170504432255455640188301913440227508544921875;0.123645279740350388930636427176068536937236785888671875;0.032365360185020501659902691926617990247905254364013671875;0.08185022997607270534015100338365300558507442474365234375;0.00571066695852551729772894617553902207873761653900146484375]
      mask Display: e = 0.06;c1 = [120 150 230]/255;c2 = ([120 150 230]+0)/383;c3 = ([120 150 230]+128)/383;patch([0 1 1 0],[0 0 1 1],c1);patch([0 1 1 1-e 1-e 0+e],[0 0 1 1-e 0+e 0+e],c2);patch([0 0 1 1-e 0+e 0+e],[0 1 1 1-e 1-e 0+e],c3);plot([0 1 1 0 0],[0 0 1 1 0]);disp('Weights');
  "IW{1,1}(58,:)'" : Constant  Value=[-0.01824907867243168169135714151707361452281475067138671875;-0.06166164488328067239120144904518383555114269256591796875;-0.060859516408848061963521303141533280722796916961669921875;0.01156026693924830893445143686903975321911275386810302734375;-0.03873897483279971354352966272927005775272846221923828125;0.07318411794400610237421034298677113838493824005126953125;-0.0012221256259491637165270905285296976217068731784820556640625;0.017284377807637009427654817272923537530004978179931640625;0.1059484592070865371926657871881616301834583282470703125;0.0016597677669346728134003310373145723133347928524017333984375]
      mask Display: e = 0.06;c1 = [120 150 230]/255;c2 = ([120 150 230]+0)/383;c3 = ([120 150 230]+128)/383;patch([0 1 1 0],[0 0 1 1],c1);patch([0 1 1 1-e 1-e 0+e],[0 0 1 1-e 0+e 0+e],c2);patch([0 0 1 1-e 0+e 0+e],[0 1 1 1-e 1-e 0+e],c3);plot([0 1 1 0 0],[0 0 1 1 0]);disp('Weights');
  "IW{1,1}(59,:)'" : Constant  Value=[0.08145697815577497558070518834938411600887775421142578125;0.0089823990285460598992361980208443128503859043121337890625;0.1029998792664417461839576617421698756515979766845703125;0.06539525364682861885423648118376149795949459075927734375;-0.0309120935822936211689881957909165066666901111602783203125;-0.076683819934392605244255491925287060439586639404296875;-0.045361471020347078619838754320880980230867862701416015625;0.01505677409928360237223454731747551704756915569305419921875;-0.1423818995820561872367449041121290065348148345947265625;0.0215879656735609680440202140516703366301953792572021484375]
      mask Display: e = 0.06;c1 = [120 150 230]/255;c2 = ([120 150 230]+0)/383;c3 = ([120 150 230]+128)/383;patch([0 1 1 0],[0 0 1 1],c1);patch([0 1 1 1-e 1-e 0+e],[0 0 1 1-e 0+e 0+e],c2);patch([0 0 1 1-e 0+e 0+e],[0 1 1 1-e 1-e 0+e],c3);plot([0 1 1 0 0],[0 0 1 1 0]);disp('Weights');
  "IW{1,1}(6,:)'" : Constant  Value=[-0.0082577866912950277644700491919138585217297077178955078125;0.1397877750083862391505817868164740502834320068359375;-0.15413928769240026195319614998879842460155487060546875;0.0216173183954049309696276992553976015187799930572509765625;0.00808739530348380648849815344192393240518867969512939453125;0.23765422014903803127339187994948588311672210693359375;0.022068581905396310316458396982852718792855739593505859375;0.01018911342714888534910500084151863120496273040771484375;0.09476845636216058021972230562823824584484100341796875;-0.00761829702490846027984616739558987319469451904296875]
      mask Display: e = 0.06;c1 = [120 150 230]/255;c2 = ([120 150 230]+0)/383;c3 = ([120 150 230]+128)/383;patch([0 1 1 0],[0 0 1 1],c1);patch([0 1 1 1-e 1-e 0+e],[0 0 1 1-e 0+e 0+e],c2);patch([0 0 1 1-e 0+e 0+e],[0 1 1 1-e 1-e 0+e],c3);plot([0 1 1 0 0],[0 0 1 1 0]);disp('Weights');
  "IW{1,1}(60,:)'" : Constant  Value=[-0.01424679127965904935904095651721945614553987979888916015625;0.0238633778440426082279035568944891565479338169097900390625;-0.026025196296788864758209314231862663291394710540771484375;0.01137565768845756782046141353248458472080528736114501953125;-0.1221770832203225298773219265058287419378757476806640625;-0.245469451159031348819183904197416268289089202880859375;-0.030097139390702125349985607272174092940986156463623046875;-0.053485790177366328290720076665820670314133167266845703125;-0.00867422841607091467397427919649999239481985569000244140625;-0.00473716975280088180288995403088847524486482143402099609375]
      mask Display: e = 0.06;c1 = [120 150 230]/255;c2 = ([120 150 230]+0)/383;c3 = ([120 150 230]+128)/383;patch([0 1 1 0],[0 0 1 1],c1);patch([0 1 1 1-e 1-e 0+e],[0 0 1 1-e 0+e 0+e],c2);patch([0 0 1 1-e 0+e 0+e],[0 1 1 1-e 1-e 0+e],c3);plot([0 1 1 0 0],[0 0 1 1 0]);disp('Weights');
  "IW{1,1}(61,:)'" : Constant  Value=[0.07407400845359705943149464246744173578917980194091796875;-0.1754665936148404881134155175459454767405986785888671875;0.044798954286753074616189707057856139726936817169189453125;-0.012215404255148276657649830667651258409023284912109375;0.0163853581189845227961132678728972678072750568389892578125;-0.135184549719042923499046082724817097187042236328125;0.07445987626175344653578491715961718000471591949462890625;0.2173724428107420558742290950249298475682735443115234375;0.021880264638977124647123417844341020099818706512451171875;0.02809248674928314926102501658533583395183086395263671875]
      mask Display: e = 0.06;c1 = [120 150 230]/255;c2 = ([120 150 230]+0)/383;c3 = ([120 150 230]+128)/383;patch([0 1 1 0],[0 0 1 1],c1);patch([0 1 1 1-e 1-e 0+e],[0 0 1 1-e 0+e 0+e],c2);patch([0 0 1 1-e 0+e 0+e],[0 1 1 1-e 1-e 0+e],c3);plot([0 1 1 0 0],[0 0 1 1 0]);disp('Weights');
  "IW{1,1}(62,:)'" : Constant  Value=[-0.01706521556266604733309577568434178829193115234375;-0.042921240827545344143079120158290606923401355743408203125;0.0250628428852150246519681076051710988394916057586669921875;-0.012985646847749089671797406708719790913164615631103515625;0.041485240536370572572710813119556405581533908843994140625;0.368636297066988138926291185271111316978931427001953125;0.092237133784504266031945007853209972381591796875;0.0149642254834280556685666141447654808871448040008544921875;0.230769066038217118830289109610021114349365234375;-8.960142623289681153048343020817156912016798742115497589111328125e-06]
      mask Display: e = 0.06;c1 = [120 150 230]/255;c2 = ([120 150 230]+0)/383;c3 = ([120 150 230]+128)/383;patch([0 1 1 0],[0 0 1 1],c1);patch([0 1 1 1-e 1-e 0+e],[0 0 1 1-e 0+e 0+e],c2);patch([0 0 1 1-e 0+e 0+e],[0 1 1 1-e 1-e 0+e],c3);plot([0 1 1 0 0],[0 0 1 1 0]);disp('Weights');
  "IW{1,1}(63,:)'" : Constant  Value=[0.047505361288316776124940332692858646623790264129638671875;-0.0121817369667278456446535273016706923954188823699951171875;0.053076786289135924334914307110011577606201171875;-0.0223821535027644465121188233069915440864861011505126953125;-0.07796885135092572471915417509080725722014904022216796875;-0.315922746886022398626892027095891535282135009765625;0.0018374603904212001050100244725626907893456518650054931640625;-0.005065411436543993360659410285506965010426938533782958984375;0.0194493232978358056295409284075503819622099399566650390625;-0.0037422351346858180598520249304783646948635578155517578125]
      mask Display: e = 0.06;c1 = [120 150 230]/255;c2 = ([120 150 230]+0)/383;c3 = ([120 150 230]+128)/383;patch([0 1 1 0],[0 0 1 1],c1);patch([0 1 1 1-e 1-e 0+e],[0 0 1 1-e 0+e 0+e],c2);patch([0 0 1 1-e 0+e 0+e],[0 1 1 1-e 1-e 0+e],c3);plot([0 1 1 0 0],[0 0 1 1 0]);disp('Weights');
  "IW{1,1}(64,:)'" : Constant  Value=[0.09721942425940925669447523205235484056174755096435546875;0.007336846033247472649574394409910382819361984729766845703125;0.22096623254027036864499677903950214385986328125;0.03714283065080610513053471777311642654240131378173828125;-0.025030470048521012704778598845223314128816127777099609375;-0.250337658351175551540990227294969372451305389404296875;0.12337313409697336918924293058807961642742156982421875;0.29262085990319908201939824721193872392177581787109375;-0.0202414639323439428386652849667370901443064212799072265625;0.031974811844667487548132811525647412054240703582763671875]
      mask Display: e = 0.06;c1 = [120 150 230]/255;c2 = ([120 150 230]+0)/383;c3 = ([120 150 230]+128)/383;patch([0 1 1 0],[0 0 1 1],c1);patch([0 1 1 1-e 1-e 0+e],[0 0 1 1-e 0+e 0+e],c2);patch([0 0 1 1-e 0+e 0+e],[0 1 1 1-e 1-e 0+e],c3);plot([0 1 1 0 0],[0 0 1 1 0]);disp('Weights');
  "IW{1,1}(65,:)'" : Constant  Value=[0.04104077586125919052673083342597237788140773773193359375;-0.0108496888498435806180708596002659760415554046630859375;0.061484883448793957450018154986537410877645015716552734375;0.028140592433979476350014437002755585126578807830810546875;0.01504213250203318384679018748784073977731168270111083984375;-0.0633240050322889935774384184696828015148639678955078125;-0.0272793943179967003642705236643450916744768619537353515625;-0.017230054951874344826290297305604326538741588592529296875;0.08609679877400455705327431132900528609752655029296875;0.005734307830445681090913989663704342092387378215789794921875]
      mask Display: e = 0.06;c1 = [120 150 230]/255;c2 = ([120 150 230]+0)/383;c3 = ([120 150 230]+128)/383;patch([0 1 1 0],[0 0 1 1],c1);patch([0 1 1 1-e 1-e 0+e],[0 0 1 1-e 0+e 0+e],c2);patch([0 0 1 1-e 0+e 0+e],[0 1 1 1-e 1-e 0+e],c3);plot([0 1 1 0 0],[0 0 1 1 0]);disp('Weights');
  "IW{1,1}(66,:)'" : Constant  Value=[0.0208543169009830949012229694972120341844856739044189453125;0.0203033349987556122062670738159795291721820831298828125;0.072183661605234428204624919089837931096553802490234375;0.033364748827921834883891705203495803289115428924560546875;0.03276741253580951751533945071059861220419406890869140625;0.3489333492505839462438643749919719994068145751953125;-0.092351893143306995614949528317083604633808135986328125;-0.02371092231740297429087860336949233897030353546142578125;0.04800147439231354506983251440033200196921825408935546875;0.020846769002330726994198784041145700030028820037841796875]
      mask Display: e = 0.06;c1 = [120 150 230]/255;c2 = ([120 150 230]+0)/383;c3 = ([120 150 230]+128)/383;patch([0 1 1 0],[0 0 1 1],c1);patch([0 1 1 1-e 1-e 0+e],[0 0 1 1-e 0+e 0+e],c2);patch([0 0 1 1-e 0+e 0+e],[0 1 1 1-e 1-e 0+e],c3);plot([0 1 1 0 0],[0 0 1 1 0]);disp('Weights');
  "IW{1,1}(67,:)'" : Constant  Value=[0.01468431322540426041400873913289615302346646785736083984375;0.07838276000018849776207474633338279090821743011474609375;0.00460774062827447837553673792854169732891023159027099609375;-0.035027021412602381278400542896633851341903209686279296875;0.0336460135799046822224767083753249607980251312255859375;0.1994266294319132770684888100731768645346164703369140625;0.12331218458196190057574170850784867070615291595458984375;-0.1401073929974854248570181880495510995388031005859375;0.061296168886501432859770233108065440319478511810302734375;-0.0030574788309185372929543955677900157752446830272674560546875]
      mask Display: e = 0.06;c1 = [120 150 230]/255;c2 = ([120 150 230]+0)/383;c3 = ([120 150 230]+128)/383;patch([0 1 1 0],[0 0 1 1],c1);patch([0 1 1 1-e 1-e 0+e],[0 0 1 1-e 0+e 0+e],c2);patch([0 0 1 1-e 0+e 0+e],[0 1 1 1-e 1-e 0+e],c3);plot([0 1 1 0 0],[0 0 1 1 0]);disp('Weights');
  "IW{1,1}(68,:)'" : Constant  Value=[-0.00801799543842561523998568873139447532594203948974609375;-0.052893017397104648280592442688430310226976871490478515625;-0.000247675787691115502180128071785247811931185424327850341796875;0.0423667645131071690656199280056171119213104248046875;-0.0101140015977881636555224531548446975648403167724609375;0.07704828157823233325540712712609092704951763153076171875;0.09363329751406047896100659500007168389856815338134765625;0.037422369688714214597258234107357566244900226593017578125;0.0201977445802810316732855966392889968119561672210693359375;-0.00811923570715679214504501004512349027208983898162841796875]
      mask Display: e = 0.06;c1 = [120 150 230]/255;c2 = ([120 150 230]+0)/383;c3 = ([120 150 230]+128)/383;patch([0 1 1 0],[0 0 1 1],c1);patch([0 1 1 1-e 1-e 0+e],[0 0 1 1-e 0+e 0+e],c2);patch([0 0 1 1-e 0+e 0+e],[0 1 1 1-e 1-e 0+e],c3);plot([0 1 1 0 0],[0 0 1 1 0]);disp('Weights');
  "IW{1,1}(69,:)'" : Constant  Value=[0.106641247842250763699922799787600524723529815673828125;0.046883227972067731403882362428703345358371734619140625;0.122437113087230653452053275032085366547107696533203125;0.06970993766294510118886051941444748081266880035400390625;-0.04704075016716617596568283943270216695964336395263671875;-0.397989990648523861427321435257908888161182403564453125;0.184822975229697317178789717218023724853992462158203125;0.29876117507895305624998627536115236580371856689453125;-0.050407286600327651238107051767656230367720127105712890625;0.01039911071588435313717280195078274118714034557342529296875]
      mask Display: e = 0.06;c1 = [120 150 230]/255;c2 = ([120 150 230]+0)/383;c3 = ([120 150 230]+128)/383;patch([0 1 1 0],[0 0 1 1],c1);patch([0 1 1 1-e 1-e 0+e],[0 0 1 1-e 0+e 0+e],c2);patch([0 0 1 1-e 0+e 0+e],[0 1 1 1-e 1-e 0+e],c3);plot([0 1 1 0 0],[0 0 1 1 0]);disp('Weights');
  "IW{1,1}(7,:)'" : Constant  Value=[0.1454101071109409615278451610720367170870304107666015625;-0.0084789699444700605823754813172854483127593994140625;0.05604335373841828893404226619168184697628021240234375;0.0303170308929605336611956545311841182410717010498046875;-0.12409623446007118918732459178499993868172168731689453125;-0.387129895738122897785871145970304496586322784423828125;0.1528241958864730298817136144862161017954349517822265625;0.216774533881226971754330179464886896312236785888671875;0.08559875122730141450144714099224074743688106536865234375;0.035793766809730488687169014383471221663057804107666015625]
      mask Display: e = 0.06;c1 = [120 150 230]/255;c2 = ([120 150 230]+0)/383;c3 = ([120 150 230]+128)/383;patch([0 1 1 0],[0 0 1 1],c1);patch([0 1 1 1-e 1-e 0+e],[0 0 1 1-e 0+e 0+e],c2);patch([0 0 1 1-e 0+e 0+e],[0 1 1 1-e 1-e 0+e],c3);plot([0 1 1 0 0],[0 0 1 1 0]);disp('Weights');
  "IW{1,1}(70,:)'" : Constant  Value=[0.0015077651940060749803651507505719564505852758884429931640625;-0.080222003285972454111885099337087012827396392822265625;0.08452370668835400280283209895060281269252300262451171875;-0.0585842197391726049460203284979797899723052978515625;-0.0029307780279438679083003904679571860469877719879150390625;0.053134495057182797028705323327812948264181613922119140625;-0.017934326798219109300180917898615007288753986358642578125;0.02038527182018175232247614303560112603008747100830078125;-0.037881831346389303882826737890354706905782222747802734375;0.0004801134016055241750427218239138937860843725502490997314453125]
      mask Display: e = 0.06;c1 = [120 150 230]/255;c2 = ([120 150 230]+0)/383;c3 = ([120 150 230]+128)/383;patch([0 1 1 0],[0 0 1 1],c1);patch([0 1 1 1-e 1-e 0+e],[0 0 1 1-e 0+e 0+e],c2);patch([0 0 1 1-e 0+e 0+e],[0 1 1 1-e 1-e 0+e],c3);plot([0 1 1 0 0],[0 0 1 1 0]);disp('Weights');
  "IW{1,1}(71,:)'" : Constant  Value=[-0.001792437619587479435967480867475387640297412872314453125;0.0134606722989981004989790136505689588375389575958251953125;-0.0112310125109178760016703790824976749718189239501953125;0.009438519071599892062973680140203214250504970550537109375;-0.05949342677782394617214123400117387063801288604736328125;-0.1021400380707226662746478496046620421111583709716796875;-0.01067127203719316942687189708749428973533213138580322265625;0.015311181301818577171758306576521135866641998291015625;0.000691578995081102462609556891237616582657210528850555419921875;-0.0011793329965906194402303075463578352355398237705230712890625]
      mask Display: e = 0.06;c1 = [120 150 230]/255;c2 = ([120 150 230]+0)/383;c3 = ([120 150 230]+128)/383;patch([0 1 1 0],[0 0 1 1],c1);patch([0 1 1 1-e 1-e 0+e],[0 0 1 1-e 0+e 0+e],c2);patch([0 0 1 1-e 0+e 0+e],[0 1 1 1-e 1-e 0+e],c3);plot([0 1 1 0 0],[0 0 1 1 0]);disp('Weights');
  "IW{1,1}(72,:)'" : Constant  Value=[0.038204255224192164297480900359005318023264408111572265625;0.1338878964639514113077467527546104975044727325439453125;0.05493371094441380775297290028902352787554264068603515625;-0.03827258716515376246736224175037932582199573516845703125;0.0927671254223006724881628315415582619607448577880859375;0.11245505584417257727292138724806136451661586761474609375;0.0949067159555107842106025373141164891421794891357421875;-0.041884687531384356962149695391417481005191802978515625;-0.08359433741168882658900685100888949818909168243408203125;0.0290343550386751615699498785261312150396406650543212890625]
      mask Display: e = 0.06;c1 = [120 150 230]/255;c2 = ([120 150 230]+0)/383;c3 = ([120 150 230]+128)/383;patch([0 1 1 0],[0 0 1 1],c1);patch([0 1 1 1-e 1-e 0+e],[0 0 1 1-e 0+e 0+e],c2);patch([0 0 1 1-e 0+e 0+e],[0 1 1 1-e 1-e 0+e],c3);plot([0 1 1 0 0],[0 0 1 1 0]);disp('Weights');
  "IW{1,1}(73,:)'" : Constant  Value=[0.01204312332081385571169729331586495391093194484710693359375;0.2110902126289757319010931269076536409556865692138671875;0.269070385021157265637015143511234782636165618896484375;0.03159457390950291821862805363707593642175197601318359375;-0.03725607436228541013978343698909156955778598785400390625;0.09014113605793112882214046521767158992588520050048828125;-0.01082760266528719032830263557798389228992164134979248046875;0.032425488617174307026669310971556114964187145233154296875;-0.137577617844151622872317375367856584489345550537109375;-0.00120847342095718561505446331238999846391379833221435546875]
      mask Display: e = 0.06;c1 = [120 150 230]/255;c2 = ([120 150 230]+0)/383;c3 = ([120 150 230]+128)/383;patch([0 1 1 0],[0 0 1 1],c1);patch([0 1 1 1-e 1-e 0+e],[0 0 1 1-e 0+e 0+e],c2);patch([0 0 1 1-e 0+e 0+e],[0 1 1 1-e 1-e 0+e],c3);plot([0 1 1 0 0],[0 0 1 1 0]);disp('Weights');
  "IW{1,1}(74,:)'" : Constant  Value=[0.006456992256854810798005761540707680978812277317047119140625;-0.056236860530816279446497674143756739795207977294921875;-0.140788603853654492592539781981031410396099090576171875;-0.0109625053256979070048782176627355511300265789031982421875;0.005873981144257412780051996747943121590651571750640869140625;0.191516130824020802680962560771149583160877227783203125;0.09446534473600311232477366729654022492468357086181640625;0.160232168936156771366086104535497725009918212890625;0.0290056528870452912105548648469266481697559356689453125;0.00096218352165836572818802263640236560604535043239593505859375]
      mask Display: e = 0.06;c1 = [120 150 230]/255;c2 = ([120 150 230]+0)/383;c3 = ([120 150 230]+128)/383;patch([0 1 1 0],[0 0 1 1],c1);patch([0 1 1 1-e 1-e 0+e],[0 0 1 1-e 0+e 0+e],c2);patch([0 0 1 1-e 0+e 0+e],[0 1 1 1-e 1-e 0+e],c3);plot([0 1 1 0 0],[0 0 1 1 0]);disp('Weights');
  "IW{1,1}(75,:)'" : Constant  Value=[0.04966615627940551558339166149380616843700408935546875;0.09639602454368932649142465152181102894246578216552734375;0.111581719356270869791813993288087658584117889404296875;0.00139661762035072994046769334630653247586451470851898193359375;-0.018028101283823046163679038045302149839699268341064453125;0.097144070015310834964594732809928245842456817626953125;-0.127601967838277430278282054132432676851749420166015625;0.0226619955242240121717767209474914125166833400726318359375;-0.1537855227005869573897456348277046345174312591552734375;0.0116768334532415807291982901006122119724750518798828125]
      mask Display: e = 0.06;c1 = [120 150 230]/255;c2 = ([120 150 230]+0)/383;c3 = ([120 150 230]+128)/383;patch([0 1 1 0],[0 0 1 1],c1);patch([0 1 1 1-e 1-e 0+e],[0 0 1 1-e 0+e 0+e],c2);patch([0 0 1 1-e 0+e 0+e],[0 1 1 1-e 1-e 0+e],c3);plot([0 1 1 0 0],[0 0 1 1 0]);disp('Weights');
  "IW{1,1}(76,:)'" : Constant  Value=[0.0355972954558171628125506913420394994318485260009765625;-0.089260926162840148467836343115777708590030670166015625;0.1124585105721112310295239922197652049362659454345703125;-0.04386939267261437402911639082958572544157505035400390625;0.11761966882812970036642497007051133550703525543212890625;0.342834617150196863111233369636465795338153839111328125;0.0726944363779905289302263327044784091413021087646484375;-0.07616810679152531682323257200550870038568973541259765625;0.066441229587955674684707219057600013911724090576171875;0.019155012939815356520778522053660708479583263397216796875]
      mask Display: e = 0.06;c1 = [120 150 230]/255;c2 = ([120 150 230]+0)/383;c3 = ([120 150 230]+128)/383;patch([0 1 1 0],[0 0 1 1],c1);patch([0 1 1 1-e 1-e 0+e],[0 0 1 1-e 0+e 0+e],c2);patch([0 0 1 1-e 0+e 0+e],[0 1 1 1-e 1-e 0+e],c3);plot([0 1 1 0 0],[0 0 1 1 0]);disp('Weights');
  "IW{1,1}(77,:)'" : Constant  Value=[0.004075618917403709025315539093980987672694027423858642578125;0.1009426386780532258757858699027565307915210723876953125;0.01525766068210547554695466487828525714576244354248046875;-0.0164033677473245965983128513698829920031130313873291015625;-0.0220448799591175421952460311558752437122166156768798828125;-0.030947954656983335530728851381354616023600101470947265625;0.000882203928591552958594912414724831251078285276889801025390625;0.04702511200969129723237216467168764211237430572509765625;0.040566873792877648774446441848340327851474285125732421875;0.0082241475689970346130142075935509637929499149322509765625]
      mask Display: e = 0.06;c1 = [120 150 230]/255;c2 = ([120 150 230]+0)/383;c3 = ([120 150 230]+128)/383;patch([0 1 1 0],[0 0 1 1],c1);patch([0 1 1 1-e 1-e 0+e],[0 0 1 1-e 0+e 0+e],c2);patch([0 0 1 1-e 0+e 0+e],[0 1 1 1-e 1-e 0+e],c3);plot([0 1 1 0 0],[0 0 1 1 0]);disp('Weights');
  "IW{1,1}(78,:)'" : Constant  Value=[-0.007757890012044942225355459441971106571145355701446533203125;-0.02819623393275137723801293532233103178441524505615234375;0.01490703906068381601190964147463091649115085601806640625;-0.034509893076210940154879835972678847610950469970703125;-0.060829346098560894973150681153128971345722675323486328125;-0.148552569017718238963965404764167033135890960693359375;0.017196265562092423462292600788714480586349964141845703125;0.08936834799846522792154956960075651295483112335205078125;-0.013308056418190765401998731931598740629851818084716796875;-0.022427001224479110874643339457179536111652851104736328125]
      mask Display: e = 0.06;c1 = [120 150 230]/255;c2 = ([120 150 230]+0)/383;c3 = ([120 150 230]+128)/383;patch([0 1 1 0],[0 0 1 1],c1);patch([0 1 1 1-e 1-e 0+e],[0 0 1 1-e 0+e 0+e],c2);patch([0 0 1 1-e 0+e 0+e],[0 1 1 1-e 1-e 0+e],c3);plot([0 1 1 0 0],[0 0 1 1 0]);disp('Weights');
  "IW{1,1}(79,:)'" : Constant  Value=[0.0267907790617882661521331755238861660473048686981201171875;0.054137894871342580327411297957951319403946399688720703125;0.021926750962385270493637534627850982360541820526123046875;-0.005900261107403721727582279754642513580620288848876953125;0.07395544609707792316211083516463986597955226898193359375;0.041715796449459836836570758578091044910252094268798828125;0.059917598899032538384279433785195578821003437042236328125;-0.12203971234138806523095155398550559766590595245361328125;0.097500826626262193652650012154481373727321624755859375;0.016615898618972411993066629065651795826852321624755859375]
      mask Display: e = 0.06;c1 = [120 150 230]/255;c2 = ([120 150 230]+0)/383;c3 = ([120 150 230]+128)/383;patch([0 1 1 0],[0 0 1 1],c1);patch([0 1 1 1-e 1-e 0+e],[0 0 1 1-e 0+e 0+e],c2);patch([0 0 1 1-e 0+e 0+e],[0 1 1 1-e 1-e 0+e],c3);plot([0 1 1 0 0],[0 0 1 1 0]);disp('Weights');
  "IW{1,1}(8,:)'" : Constant  Value=[0.01518355032274369686984272220797720365226268768310546875;-0.049878370475438839337645191562842228449881076812744140625;-0.08823249605939890993777652283824863843619823455810546875;0.0145340345051295505296451437970972619950771331787109375;-0.0047150587134948927781064043074366054497659206390380859375;0.300003002422858877640265973241184838116168975830078125;-0.032509512699926045031784127559149055741727352142333984375;-0.019315091521401039909022756546619348227977752685546875;0.1679337264908744298264053895763936452567577362060546875;0.0148231174893603302733513515931917936541140079498291015625]
      mask Display: e = 0.06;c1 = [120 150 230]/255;c2 = ([120 150 230]+0)/383;c3 = ([120 150 230]+128)/383;patch([0 1 1 0],[0 0 1 1],c1);patch([0 1 1 1-e 1-e 0+e],[0 0 1 1-e 0+e 0+e],c2);patch([0 0 1 1-e 0+e 0+e],[0 1 1 1-e 1-e 0+e],c3);plot([0 1 1 0 0],[0 0 1 1 0]);disp('Weights');
  "IW{1,1}(80,:)'" : Constant  Value=[0.0060923368396083067699553481588736758567392826080322265625;0.10190297567157798053205652877295506186783313751220703125;0.042024578510304173850631315190184977836906909942626953125;-0.0106047564104820336849943629431436420418322086334228515625;0.003865069927908253329118526409047262859530746936798095703125;0.2269617277767885521466695308845373801887035369873046875;0.0028525565780745110178173717940808273851871490478515625;0.0262292333878444694494902478254516609013080596923828125;0.15012411816246717943812427620287053287029266357421875;0.01310972686983256051129753672057631774805486202239990234375]
      mask Display: e = 0.06;c1 = [120 150 230]/255;c2 = ([120 150 230]+0)/383;c3 = ([120 150 230]+128)/383;patch([0 1 1 0],[0 0 1 1],c1);patch([0 1 1 1-e 1-e 0+e],[0 0 1 1-e 0+e 0+e],c2);patch([0 0 1 1-e 0+e 0+e],[0 1 1 1-e 1-e 0+e],c3);plot([0 1 1 0 0],[0 0 1 1 0]);disp('Weights');
  "IW{1,1}(81,:)'" : Constant  Value=[0.12198127490235648184846439789907890371978282928466796875;-0.03820173417653005554228684559348039329051971435546875;-0.0291214753516970716040734856733251945115625858306884765625;-0.00826449763578827011067939878330435021780431270599365234375;0.0238631026303488813500308651782688684761524200439453125;-0.10446593650549949872097243996904580853879451751708984375;0.1861941280775017693027706400243914686143398284912109375;-0.139662826890534663704102058545686304569244384765625;0.03836549303000945376762587102348334155976772308349609375;0.025204460544893982076875005304827936924993991851806640625]
      mask Display: e = 0.06;c1 = [120 150 230]/255;c2 = ([120 150 230]+0)/383;c3 = ([120 150 230]+128)/383;patch([0 1 1 0],[0 0 1 1],c1);patch([0 1 1 1-e 1-e 0+e],[0 0 1 1-e 0+e 0+e],c2);patch([0 0 1 1-e 0+e 0+e],[0 1 1 1-e 1-e 0+e],c3);plot([0 1 1 0 0],[0 0 1 1 0]);disp('Weights');
  "IW{1,1}(82,:)'" : Constant  Value=[-0.004231996909069086522381386572533301659859716892242431640625;0.01106062088632323893444553419840303831733763217926025390625;-0.0104355866325197867150453845397350960411131381988525390625;-0.0038639520518201487912779423794518152135424315929412841796875;-0.048771332492827161597670482251487555913627147674560546875;-0.0945485572081659897403227432732819579541683197021484375;-0.01077079925954782697872236241209975560195744037628173828125;0.01217014211873092277560459706364781595766544342041015625;0.000952098700140476157660618383715700474567711353302001953125;-0.0023051874232068261284800403387862388626672327518463134765625]
      mask Display: e = 0.06;c1 = [120 150 230]/255;c2 = ([120 150 230]+0)/383;c3 = ([120 150 230]+128)/383;patch([0 1 1 0],[0 0 1 1],c1);patch([0 1 1 1-e 1-e 0+e],[0 0 1 1-e 0+e 0+e],c2);patch([0 0 1 1-e 0+e 0+e],[0 1 1 1-e 1-e 0+e],c3);plot([0 1 1 0 0],[0 0 1 1 0]);disp('Weights');
  "IW{1,1}(83,:)'" : Constant  Value=[0.113894568641141058495946936091058887541294097900390625;-0.1324292155592957931364850310274050571024417877197265625;-0.049489726174868853281196834359434433281421661376953125;-0.0293649136190072233831838133255587308667600154876708984375;-0.034160087179264726764404969117094879038631916046142578125;-0.1952286500896077969802178131430991925299167633056640625;-0.00977017384912916286854311920251348055899143218994140625;0.0108934788822734086866095282175592728890478610992431640625;-0.0303244750455853410986417628691924619488418102264404296875;0.01152199525290467131688476598583292798139154911041259765625]
      mask Display: e = 0.06;c1 = [120 150 230]/255;c2 = ([120 150 230]+0)/383;c3 = ([120 150 230]+128)/383;patch([0 1 1 0],[0 0 1 1],c1);patch([0 1 1 1-e 1-e 0+e],[0 0 1 1-e 0+e 0+e],c2);patch([0 0 1 1-e 0+e 0+e],[0 1 1 1-e 1-e 0+e],c3);plot([0 1 1 0 0],[0 0 1 1 0]);disp('Weights');
  "IW{1,1}(84,:)'" : Constant  Value=[0.0717184464613162264701173853609361685812473297119140625;0.03983698090799238367143431105432682670652866363525390625;0.1417012765698767162714233336373581551015377044677734375;0.0168551838377525887990859843057478428818285465240478515625;0.00967633539370988011996121969104933668859302997589111328125;-0.157281562885221937175828088584239594638347625732421875;-0.06706005438991020917161023362496052868664264678955078125;0.061464320162308426487296486584455124102532863616943359375;0.00653474229222887614820791668535093776881694793701171875;0.01235045487037114524120351433111864025704562664031982421875]
      mask Display: e = 0.06;c1 = [120 150 230]/255;c2 = ([120 150 230]+0)/383;c3 = ([120 150 230]+128)/383;patch([0 1 1 0],[0 0 1 1],c1);patch([0 1 1 1-e 1-e 0+e],[0 0 1 1-e 0+e 0+e],c2);patch([0 0 1 1-e 0+e 0+e],[0 1 1 1-e 1-e 0+e],c3);plot([0 1 1 0 0],[0 0 1 1 0]);disp('Weights');
  "IW{1,1}(85,:)'" : Constant  Value=[0.0667692104304247191493004720541648566722869873046875;-0.0185627916265010683982694672522484324872493743896484375;0.08708630401798629627752035275989328511059284210205078125;-0.0170063986077842142774496636548064998351037502288818359375;0.04204854563584790871910712439785129390656948089599609375;-0.0615355226255117904177183163483277894556522369384765625;0.036053576512514694252242719585410668514668941497802734375;0.1863601366955400795433206440065987408161163330078125;-0.1312798630335631766552495491851004771888256072998046875;0.0166327410626927289782894803238377789966762065887451171875]
      mask Display: e = 0.06;c1 = [120 150 230]/255;c2 = ([120 150 230]+0)/383;c3 = ([120 150 230]+128)/383;patch([0 1 1 0],[0 0 1 1],c1);patch([0 1 1 1-e 1-e 0+e],[0 0 1 1-e 0+e 0+e],c2);patch([0 0 1 1-e 0+e 0+e],[0 1 1 1-e 1-e 0+e],c3);plot([0 1 1 0 0],[0 0 1 1 0]);disp('Weights');
  "IW{1,1}(86,:)'" : Constant  Value=[-0.00961854802860433004407791912626635166816413402557373046875;-0.02622834602841488116364843108385684899985790252685546875;0.01386941824325689520680526811702293343842029571533203125;-0.0575319078384433080231019630446098744869232177734375;-0.004837626953600044667214152838141671963967382907867431640625;-0.056612913096742233098890295650562620721757411956787109375;0.047913767234589170473935126892683911137282848358154296875;-0.0289640904004426803786120814265814260579645633697509765625;-0.005490894873670051738734354529469783301465213298797607421875;-0.0178505581291122754350464418848787317983806133270263671875]
      mask Display: e = 0.06;c1 = [120 150 230]/255;c2 = ([120 150 230]+0)/383;c3 = ([120 150 230]+128)/383;patch([0 1 1 0],[0 0 1 1],c1);patch([0 1 1 1-e 1-e 0+e],[0 0 1 1-e 0+e 0+e],c2);patch([0 0 1 1-e 0+e 0+e],[0 1 1 1-e 1-e 0+e],c3);plot([0 1 1 0 0],[0 0 1 1 0]);disp('Weights');
  "IW{1,1}(87,:)'" : Constant  Value=[0.01086849862414028707047197741530908388085663318634033203125;-0.0797842554471249465475324313956662081182003021240234375;0.071014964620141951545662095668376423418521881103515625;-0.02287954182402585079358914299518801271915435791015625;0.032373706859717361894457354765108902938663959503173828125;0.1049205000110931818024795347810140810906887054443359375;0.006884937492768716284230468005489456118084490299224853515625;0.1002791979221617502116004061463172547519207000732421875;-0.00735059610793221442082145955509986379183828830718994140625;0.00828842416188708096258519475441062240861356258392333984375]
      mask Display: e = 0.06;c1 = [120 150 230]/255;c2 = ([120 150 230]+0)/383;c3 = ([120 150 230]+128)/383;patch([0 1 1 0],[0 0 1 1],c1);patch([0 1 1 1-e 1-e 0+e],[0 0 1 1-e 0+e 0+e],c2);patch([0 0 1 1-e 0+e 0+e],[0 1 1 1-e 1-e 0+e],c3);plot([0 1 1 0 0],[0 0 1 1 0]);disp('Weights');
  "IW{1,1}(88,:)'" : Constant  Value=[0.051517845824200443616280864489453961141407489776611328125;0.044753741220294969427317965937618282623589038848876953125;-0.01558139772335692153915065460978439659811556339263916015625;0.0082469766797734871122127486842146026901900768280029296875;-0.0285102437053763833885167144899241975508630275726318359375;-0.07828083815015333957187948499267804436385631561279296875;-0.0306782767671126381514579151144062052480876445770263671875;-0.034361201383013677268518648588724317960441112518310546875;0.157015139608656262293351346670533530414104461669921875;0.010555167713106779203702245695239980705082416534423828125]
      mask Display: e = 0.06;c1 = [120 150 230]/255;c2 = ([120 150 230]+0)/383;c3 = ([120 150 230]+128)/383;patch([0 1 1 0],[0 0 1 1],c1);patch([0 1 1 1-e 1-e 0+e],[0 0 1 1-e 0+e 0+e],c2);patch([0 0 1 1-e 0+e 0+e],[0 1 1 1-e 1-e 0+e],c3);plot([0 1 1 0 0],[0 0 1 1 0]);disp('Weights');
  "IW{1,1}(89,:)'" : Constant  Value=[0.056812625142005523937172029036446474492549896240234375;0.15903135975361759602009215086582116782665252685546875;0.07201653173913032113251375676554744131863117218017578125;0.03312683986816224168681088713128701783716678619384765625;-0.06155112675022915424971614584137569181621074676513671875;0.09099664784385808058431166500668041408061981201171875;-0.156148544380291076638656022623763419687747955322265625;-0.11859048700056627756449501021052128635346889495849609375;0.027217195004993373352863983427596394903957843780517578125;0.0249204535234069067539675046418778947554528713226318359375]
      mask Display: e = 0.06;c1 = [120 150 230]/255;c2 = ([120 150 230]+0)/383;c3 = ([120 150 230]+128)/383;patch([0 1 1 0],[0 0 1 1],c1);patch([0 1 1 1-e 1-e 0+e],[0 0 1 1-e 0+e 0+e],c2);patch([0 0 1 1-e 0+e 0+e],[0 1 1 1-e 1-e 0+e],c3);plot([0 1 1 0 0],[0 0 1 1 0]);disp('Weights');
  "IW{1,1}(9,:)'" : Constant  Value=[0.01709887410587933309624730782161350362002849578857421875;-0.05854452939737249395069085267095942981541156768798828125;-0.12581699412104629942632527672685682773590087890625;0.0384023549572090339143670689736609347164630889892578125;-0.03813343541399068226116497726252418942749500274658203125;0.10494511358365442299511727242133929394185543060302734375;0.1113841087411903407744517835453734733164310455322265625;-0.0399061863962293650320845017631654627621173858642578125;0.11018377717862924691782922081983997486531734466552734375;0.005006549323405479375026505550749789108522236347198486328125]
      mask Display: e = 0.06;c1 = [120 150 230]/255;c2 = ([120 150 230]+0)/383;c3 = ([120 150 230]+128)/383;patch([0 1 1 0],[0 0 1 1],c1);patch([0 1 1 1-e 1-e 0+e],[0 0 1 1-e 0+e 0+e],c2);patch([0 0 1 1-e 0+e 0+e],[0 1 1 1-e 1-e 0+e],c3);plot([0 1 1 0 0],[0 0 1 1 0]);disp('Weights');
  "IW{1,1}(90,:)'" : Constant  Value=[0.02169827918873636074525990125039243139326572418212890625;-0.07248089766536469635838102476554922759532928466796875;-0.04521466864739571989151301067977328784763813018798828125;0.01141941353659275439069720192719614715315401554107666015625;0.036757161446345006095004492863154155202209949493408203125;0.10026315538967123242031220797798596322536468505859375;0.049904019266024009227056268400701810605823993682861328125;0.1826485330990869904166373771658982150256633758544921875;-0.116217750714762979580285673364414833486080169677734375;0.005745324519992754154495973040184253477491438388824462890625]
      mask Display: e = 0.06;c1 = [120 150 230]/255;c2 = ([120 150 230]+0)/383;c3 = ([120 150 230]+128)/383;patch([0 1 1 0],[0 0 1 1],c1);patch([0 1 1 1-e 1-e 0+e],[0 0 1 1-e 0+e 0+e],c2);patch([0 0 1 1-e 0+e 0+e],[0 1 1 1-e 1-e 0+e],c3);plot([0 1 1 0 0],[0 0 1 1 0]);disp('Weights');
  "IW{1,1}(91,:)'" : Constant  Value=[0.12783428474476699054918071851716376841068267822265625;0.081984448846170454583415221350151114165782928466796875;0.06361927604771257238613912932123639620840549468994140625;0.10669427707259504511938530413317494094371795654296875;-0.1473887583856564875706141037881025113165378570556640625;-0.251643321062409663912973201149725355207920074462890625;0.0290502834515634460188504561983791063539683818817138671875;0.035818798438621325674890982782017090357840061187744140625;-0.0258063561798649900025370840239702374674379825592041015625;0.032210541182704881257858886556277866475284099578857421875]
      mask Display: e = 0.06;c1 = [120 150 230]/255;c2 = ([120 150 230]+0)/383;c3 = ([120 150 230]+128)/383;patch([0 1 1 0],[0 0 1 1],c1);patch([0 1 1 1-e 1-e 0+e],[0 0 1 1-e 0+e 0+e],c2);patch([0 0 1 1-e 0+e 0+e],[0 1 1 1-e 1-e 0+e],c3);plot([0 1 1 0 0],[0 0 1 1 0]);disp('Weights');
  "IW{1,1}(92,:)'" : Constant  Value=[0.00421896219651842450948375784491872764192521572113037109375;0.0740114658544792636263309759669937193393707275390625;-0.035079160757796316871814923388228635303676128387451171875;-0.0260924028833688821660263812418634188361465930938720703125;0.09660111574426377689661649128538556396961212158203125;0.32077397668604767932976074007456190884113311767578125;0.09092559466424911251980489623747416771948337554931640625;-0.03580942097310384208963540686454507522284984588623046875;0.1713101540590659943585905011786962859332561492919921875;0.01820782173644942825152526211240910924971103668212890625]
      mask Display: e = 0.06;c1 = [120 150 230]/255;c2 = ([120 150 230]+0)/383;c3 = ([120 150 230]+128)/383;patch([0 1 1 0],[0 0 1 1],c1);patch([0 1 1 1-e 1-e 0+e],[0 0 1 1-e 0+e 0+e],c2);patch([0 0 1 1-e 0+e 0+e],[0 1 1 1-e 1-e 0+e],c3);plot([0 1 1 0 0],[0 0 1 1 0]);disp('Weights');
  "IW{1,1}(93,:)'" : Constant  Value=[-0.0021832166599717955056403351221661068848334252834320068359375;0.004790178314980118347288229330160902463831007480621337890625;-0.0052755658866645745164181136033221264369785785675048828125;0.0028699918061751632063216543855332929524593055248260498046875;-0.0206747156283349532712723117811037809588015079498291015625;-0.036083802452121387094319260313568520359694957733154296875;-0.00455868247668037886166647609798019402660429477691650390625;0.005175581570914658709192668339937881682999432086944580078125;-0.0003058588685547932437859552923242745237075723707675933837890625;-0.00107881132001048343944937801808237054501660168170928955078125]
      mask Display: e = 0.06;c1 = [120 150 230]/255;c2 = ([120 150 230]+0)/383;c3 = ([120 150 230]+128)/383;patch([0 1 1 0],[0 0 1 1],c1);patch([0 1 1 1-e 1-e 0+e],[0 0 1 1-e 0+e 0+e],c2);patch([0 0 1 1-e 0+e 0+e],[0 1 1 1-e 1-e 0+e],c3);plot([0 1 1 0 0],[0 0 1 1 0]);disp('Weights');
  "IW{1,1}(94,:)'" : Constant  Value=[0.0336929853820808478115367279315250925719738006591796875;0.214314278798693080840820357479969970881938934326171875;0.031823668049836141558106561433305614627897739410400390625;-0.027470141505335853027158776740179746411740779876708984375;0.144140871100235823387691880270722322165966033935546875;0.08107086550394097812510807443686644546687602996826171875;0.049776066756170654625801574866272858344018459320068359375;-0.0108015601055814862430093370448958012275397777557373046875;0.0768540248813767978841582362292683683335781097412109375;0.0290259867463955288646726415890952921472489833831787109375]
      mask Display: e = 0.06;c1 = [120 150 230]/255;c2 = ([120 150 230]+0)/383;c3 = ([120 150 230]+128)/383;patch([0 1 1 0],[0 0 1 1],c1);patch([0 1 1 1-e 1-e 0+e],[0 0 1 1-e 0+e 0+e],c2);patch([0 0 1 1-e 0+e 0+e],[0 1 1 1-e 1-e 0+e],c3);plot([0 1 1 0 0],[0 0 1 1 0]);disp('Weights');
  "IW{1,1}(95,:)'" : Constant  Value=[0.053362433855857739628536506870659650303423404693603515625;0.09471490817111354043600357499599340371787548065185546875;-0.147294733665045474158006300058332271873950958251953125;0.01230156139613267952948039152261117123998701572418212890625;-0.032236988227514147553609547003361512906849384307861328125;0.11038774851603150306544876002590171992778778076171875;-0.0169309835017730052342255220310107688419520854949951171875;0.01532161029929292143936248038471603649668395519256591796875;0.054805790222098860198229886009357869625091552734375;0.0089683339186607084758673380520122009329497814178466796875]
      mask Display: e = 0.06;c1 = [120 150 230]/255;c2 = ([120 150 230]+0)/383;c3 = ([120 150 230]+128)/383;patch([0 1 1 0],[0 0 1 1],c1);patch([0 1 1 1-e 1-e 0+e],[0 0 1 1-e 0+e 0+e],c2);patch([0 0 1 1-e 0+e 0+e],[0 1 1 1-e 1-e 0+e],c3);plot([0 1 1 0 0],[0 0 1 1 0]);disp('Weights');
  "IW{1,1}(96,:)'" : Constant  Value=[0.01069130918643866091921612593296231352724134922027587890625;-0.0162907576046158152072163005641414201818406581878662109375;0.0213174580243236273802143188049740274436771869659423828125;-0.0264404435101541594732577067361489753238856792449951171875;-0.07098437574746642442224953128970810212194919586181640625;-0.1614402258198352202445136072128661908209323883056640625;-0.01223818189886543249256245502465390018187463283538818359375;0.0091504285956384538713859200242950464598834514617919921875;-0.000176668608753232335428773325247675529681146144866943359375;-0.00121402126152318876224633914517880839412100613117218017578125]
      mask Display: e = 0.06;c1 = [120 150 230]/255;c2 = ([120 150 230]+0)/383;c3 = ([120 150 230]+128)/383;patch([0 1 1 0],[0 0 1 1],c1);patch([0 1 1 1-e 1-e 0+e],[0 0 1 1-e 0+e 0+e],c2);patch([0 0 1 1-e 0+e 0+e],[0 1 1 1-e 1-e 0+e],c3);plot([0 1 1 0 0],[0 0 1 1 0]);disp('Weights');
  "IW{1,1}(97,:)'" : Constant  Value=[0.03250138085528331277629376927507109940052032470703125;-0.040032682798133316370847722964754211716353893280029296875;-0.01353651001158347362551825909804392722435295581817626953125;-0.00625283212249686838613005335218986147083342075347900390625;0.0548493030789656554890854067707550711929798126220703125;0.2247235639508279592124750934090116061270236968994140625;0.052699819848429273194678756908615469001233577728271484375;-0.047666851053331078802433040664254804141819477081298828125;-0.07619309048928353533813861986345727927982807159423828125;0.0277462760715122928878439978461756254546344280242919921875]
      mask Display: e = 0.06;c1 = [120 150 230]/255;c2 = ([120 150 230]+0)/383;c3 = ([120 150 230]+128)/383;patch([0 1 1 0],[0 0 1 1],c1);patch([0 1 1 1-e 1-e 0+e],[0 0 1 1-e 0+e 0+e],c2);patch([0 0 1 1-e 0+e 0+e],[0 1 1 1-e 1-e 0+e],c3);plot([0 1 1 0 0],[0 0 1 1 0]);disp('Weights');
  "IW{1,1}(98,:)'" : Constant  Value=[0.03779283361975392663278938698567799292504787445068359375;-0.08463373773043626757672797111808904446661472320556640625;-0.12182633321566989359485688737549935467541217803955078125;0.00215928753565482710319312076308051473461091518402099609375;0.04099615320571314835973453227779828011989593505859375;0.04428608774707114281721231918709236197173595428466796875;0.053717522024567809779682647786103188991546630859375;0.004205893302312142811860695701398071832954883575439453125;-0.002323835929066043505530902990585673251189291477203369140625;0.0364006308049105997692862501935451291501522064208984375]
      mask Display: e = 0.06;c1 = [120 150 230]/255;c2 = ([120 150 230]+0)/383;c3 = ([120 150 230]+128)/383;patch([0 1 1 0],[0 0 1 1],c1);patch([0 1 1 1-e 1-e 0+e],[0 0 1 1-e 0+e 0+e],c2);patch([0 0 1 1-e 0+e 0+e],[0 1 1 1-e 1-e 0+e],c3);plot([0 1 1 0 0],[0 0 1 1 0]);disp('Weights');
  "IW{1,1}(99,:)'" : Constant  Value=[0.05222446281219821073715792181246797554194927215576171875;-0.076090179638263089056948729194118641316890716552734375;-0.10629333019203658639018073017723509110510349273681640625;0.022505670948543797516006037540137185715138912200927734375;-0.01183824250620214672824470625300818937830626964569091796875;0.11959831565918817297689002998595242388546466827392578125;0.03338918262165646577699362751445733010768890380859375;-0.0080914877254339954981698923575095250271260738372802734375;-0.02614553895921910287025724528575665317475795745849609375;0.0038675777705638558594258835654500217060558497905731201171875]
      mask Display: e = 0.06;c1 = [120 150 230]/255;c2 = ([120 150 230]+0)/383;c3 = ([120 150 230]+128)/383;patch([0 1 1 0],[0 0 1 1],c1);patch([0 1 1 1-e 1-e 0+e],[0 0 1 1-e 0+e 0+e],c2);patch([0 0 1 1-e 0+e 0+e],[0 1 1 1-e 1-e 0+e],c3);plot([0 1 1 0 0],[0 0 1 1 0]);disp('Weights');
  Mux : Mux  Inputs=100
      mask Display: e = 0.06;c1 = [120 150 230]/255;c2 = ([120 150 230]+0)/383;c3 = ([120 150 230]+128)/383;patch([0 1 1 0],[0 0 1 1],c1);patch([0 1 1 1-e 1-e 0+e],[0 0 1 1-e 0+e 0+e],c2);patch([0 0 1 1-e 0+e 0+e],[0 1 1 1-e 1-e 0+e],c3);plot([0 1 1 0 0],[0 0 1 1 0]);disp('Mux');
  dotprod{1..100} (100 alike) : neural/Weight Functions/dotprod
  "iz{1,1}" : Outport
      mask Display: e = 0.06;c1 = [120 230 180]/255;c2 = ([120 230 180]+0)/(256+128);c3 = ([120 230 180]+128)/(256+128);patch([0 1 1 0],[0 0 1 1],c1);patch([0 1 1 1-e 1-e 0+e],[0 0 1 1-e 0+e 0+e],c2);patch([0 0 1 1-e 0+e 0+e],[0 1 1 1-e 1-e 0+e],c3);plot([0 1 1 0 0],[0 0 1 1 0]);
  wires:
  Mux/1 -> "iz{1,1}"/1
  dotprod100/1 -> Mux/100
  "IW{1,1}(100,:)'"/1 -> dotprod100/1
  dotprod99/1 -> Mux/99
  "IW{1,1}(99,:)'"/1 -> dotprod99/1
  dotprod98/1 -> Mux/98
  "IW{1,1}(98,:)'"/1 -> dotprod98/1
  dotprod97/1 -> Mux/97
  "IW{1,1}(97,:)'"/1 -> dotprod97/1
  dotprod96/1 -> Mux/96
  "IW{1,1}(96,:)'"/1 -> dotprod96/1
  dotprod95/1 -> Mux/95
  "IW{1,1}(95,:)'"/1 -> dotprod95/1
  dotprod94/1 -> Mux/94
  "IW{1,1}(94,:)'"/1 -> dotprod94/1
  dotprod93/1 -> Mux/93
  "IW{1,1}(93,:)'"/1 -> dotprod93/1
  dotprod92/1 -> Mux/92
  "IW{1,1}(92,:)'"/1 -> dotprod92/1
  dotprod91/1 -> Mux/91
  "IW{1,1}(91,:)'"/1 -> dotprod91/1
  dotprod90/1 -> Mux/90
  "IW{1,1}(90,:)'"/1 -> dotprod90/1
  dotprod89/1 -> Mux/89
  "IW{1,1}(89,:)'"/1 -> dotprod89/1
  dotprod88/1 -> Mux/88
  "IW{1,1}(88,:)'"/1 -> dotprod88/1
  dotprod87/1 -> Mux/87
  "IW{1,1}(87,:)'"/1 -> dotprod87/1
  dotprod86/1 -> Mux/86
  "IW{1,1}(86,:)'"/1 -> dotprod86/1
  dotprod85/1 -> Mux/85
  "IW{1,1}(85,:)'"/1 -> dotprod85/1
  dotprod84/1 -> Mux/84
  "IW{1,1}(84,:)'"/1 -> dotprod84/1
  dotprod83/1 -> Mux/83
  "IW{1,1}(83,:)'"/1 -> dotprod83/1
  dotprod82/1 -> Mux/82
  "IW{1,1}(82,:)'"/1 -> dotprod82/1
  dotprod81/1 -> Mux/81
  "IW{1,1}(81,:)'"/1 -> dotprod81/1
  dotprod80/1 -> Mux/80
  "IW{1,1}(80,:)'"/1 -> dotprod80/1
  dotprod79/1 -> Mux/79
  "IW{1,1}(79,:)'"/1 -> dotprod79/1
  dotprod78/1 -> Mux/78
  "IW{1,1}(78,:)'"/1 -> dotprod78/1
  dotprod77/1 -> Mux/77
  "IW{1,1}(77,:)'"/1 -> dotprod77/1
  dotprod76/1 -> Mux/76
  "IW{1,1}(76,:)'"/1 -> dotprod76/1
  dotprod75/1 -> Mux/75
  "IW{1,1}(75,:)'"/1 -> dotprod75/1
  dotprod74/1 -> Mux/74
  "IW{1,1}(74,:)'"/1 -> dotprod74/1
  dotprod73/1 -> Mux/73
  "IW{1,1}(73,:)'"/1 -> dotprod73/1
  dotprod72/1 -> Mux/72
  "IW{1,1}(72,:)'"/1 -> dotprod72/1
  dotprod71/1 -> Mux/71
  "IW{1,1}(71,:)'"/1 -> dotprod71/1
  dotprod70/1 -> Mux/70
  "IW{1,1}(70,:)'"/1 -> dotprod70/1
  dotprod69/1 -> Mux/69
  "IW{1,1}(69,:)'"/1 -> dotprod69/1
  dotprod68/1 -> Mux/68
  "IW{1,1}(68,:)'"/1 -> dotprod68/1
  dotprod67/1 -> Mux/67
  "IW{1,1}(67,:)'"/1 -> dotprod67/1
  dotprod66/1 -> Mux/66
  "IW{1,1}(66,:)'"/1 -> dotprod66/1
  dotprod65/1 -> Mux/65
  "IW{1,1}(65,:)'"/1 -> dotprod65/1
  dotprod64/1 -> Mux/64
  "IW{1,1}(64,:)'"/1 -> dotprod64/1
  dotprod63/1 -> Mux/63
  "IW{1,1}(63,:)'"/1 -> dotprod63/1
  dotprod62/1 -> Mux/62
  "IW{1,1}(62,:)'"/1 -> dotprod62/1
  dotprod61/1 -> Mux/61
  "IW{1,1}(61,:)'"/1 -> dotprod61/1
  dotprod60/1 -> Mux/60
  "IW{1,1}(60,:)'"/1 -> dotprod60/1
  dotprod59/1 -> Mux/59
  "IW{1,1}(59,:)'"/1 -> dotprod59/1
  dotprod58/1 -> Mux/58
  "IW{1,1}(58,:)'"/1 -> dotprod58/1
  dotprod57/1 -> Mux/57
  "IW{1,1}(57,:)'"/1 -> dotprod57/1
  dotprod56/1 -> Mux/56
  "IW{1,1}(56,:)'"/1 -> dotprod56/1
  dotprod55/1 -> Mux/55
  "IW{1,1}(55,:)'"/1 -> dotprod55/1
  dotprod54/1 -> Mux/54
  "IW{1,1}(54,:)'"/1 -> dotprod54/1
  dotprod53/1 -> Mux/53
  "IW{1,1}(53,:)'"/1 -> dotprod53/1
  dotprod52/1 -> Mux/52
  "IW{1,1}(52,:)'"/1 -> dotprod52/1
  dotprod51/1 -> Mux/51
  "IW{1,1}(51,:)'"/1 -> dotprod51/1
  dotprod50/1 -> Mux/50
  "IW{1,1}(50,:)'"/1 -> dotprod50/1
  dotprod49/1 -> Mux/49
  "IW{1,1}(49,:)'"/1 -> dotprod49/1
  dotprod48/1 -> Mux/48
  "IW{1,1}(48,:)'"/1 -> dotprod48/1
  dotprod47/1 -> Mux/47
  "IW{1,1}(47,:)'"/1 -> dotprod47/1
  dotprod46/1 -> Mux/46
  "IW{1,1}(46,:)'"/1 -> dotprod46/1
  dotprod45/1 -> Mux/45
  "IW{1,1}(45,:)'"/1 -> dotprod45/1
  dotprod44/1 -> Mux/44
  "IW{1,1}(44,:)'"/1 -> dotprod44/1
  dotprod43/1 -> Mux/43
  "IW{1,1}(43,:)'"/1 -> dotprod43/1
  dotprod42/1 -> Mux/42
  "IW{1,1}(42,:)'"/1 -> dotprod42/1
  dotprod41/1 -> Mux/41
  "IW{1,1}(41,:)'"/1 -> dotprod41/1
  dotprod40/1 -> Mux/40
  "IW{1,1}(40,:)'"/1 -> dotprod40/1
  dotprod39/1 -> Mux/39
  "IW{1,1}(39,:)'"/1 -> dotprod39/1
  dotprod38/1 -> Mux/38
  "IW{1,1}(38,:)'"/1 -> dotprod38/1
  dotprod37/1 -> Mux/37
  "IW{1,1}(37,:)'"/1 -> dotprod37/1
  dotprod36/1 -> Mux/36
  "IW{1,1}(36,:)'"/1 -> dotprod36/1
  dotprod35/1 -> Mux/35
  "IW{1,1}(35,:)'"/1 -> dotprod35/1
  dotprod34/1 -> Mux/34
  "IW{1,1}(34,:)'"/1 -> dotprod34/1
  dotprod33/1 -> Mux/33
  "IW{1,1}(33,:)'"/1 -> dotprod33/1
  dotprod32/1 -> Mux/32
  "IW{1,1}(32,:)'"/1 -> dotprod32/1
  dotprod31/1 -> Mux/31
  "IW{1,1}(31,:)'"/1 -> dotprod31/1
  dotprod30/1 -> Mux/30
  "IW{1,1}(30,:)'"/1 -> dotprod30/1
  dotprod29/1 -> Mux/29
  "IW{1,1}(29,:)'"/1 -> dotprod29/1
  dotprod28/1 -> Mux/28
  "IW{1,1}(28,:)'"/1 -> dotprod28/1
  dotprod27/1 -> Mux/27
  "IW{1,1}(27,:)'"/1 -> dotprod27/1
  dotprod26/1 -> Mux/26
  "IW{1,1}(26,:)'"/1 -> dotprod26/1
  dotprod25/1 -> Mux/25
  "IW{1,1}(25,:)'"/1 -> dotprod25/1
  dotprod24/1 -> Mux/24
  "IW{1,1}(24,:)'"/1 -> dotprod24/1
  dotprod23/1 -> Mux/23
  "IW{1,1}(23,:)'"/1 -> dotprod23/1
  dotprod22/1 -> Mux/22
  "IW{1,1}(22,:)'"/1 -> dotprod22/1
  dotprod21/1 -> Mux/21
  "IW{1,1}(21,:)'"/1 -> dotprod21/1
  dotprod20/1 -> Mux/20
  "IW{1,1}(20,:)'"/1 -> dotprod20/1
  dotprod19/1 -> Mux/19
  "IW{1,1}(19,:)'"/1 -> dotprod19/1
  dotprod18/1 -> Mux/18
  "IW{1,1}(18,:)'"/1 -> dotprod18/1
  dotprod17/1 -> Mux/17
  "IW{1,1}(17,:)'"/1 -> dotprod17/1
  dotprod16/1 -> Mux/16
  "IW{1,1}(16,:)'"/1 -> dotprod16/1
  dotprod15/1 -> Mux/15
  "IW{1,1}(15,:)'"/1 -> dotprod15/1
  dotprod14/1 -> Mux/14
  "IW{1,1}(14,:)'"/1 -> dotprod14/1
  dotprod13/1 -> Mux/13
  "IW{1,1}(13,:)'"/1 -> dotprod13/1
  dotprod12/1 -> Mux/12
  "IW{1,1}(12,:)'"/1 -> dotprod12/1
  dotprod11/1 -> Mux/11
  "IW{1,1}(11,:)'"/1 -> dotprod11/1
  dotprod10/1 -> Mux/10
  "IW{1,1}(10,:)'"/1 -> dotprod10/1
  dotprod9/1 -> Mux/9
  "IW{1,1}(9,:)'"/1 -> dotprod9/1
  dotprod8/1 -> Mux/8
  "IW{1,1}(8,:)'"/1 -> dotprod8/1
  dotprod7/1 -> Mux/7
  "IW{1,1}(7,:)'"/1 -> dotprod7/1
  dotprod6/1 -> Mux/6
  "IW{1,1}(6,:)'"/1 -> dotprod6/1
  dotprod5/1 -> Mux/5
  "IW{1,1}(5,:)'"/1 -> dotprod5/1
  dotprod4/1 -> Mux/4
  "IW{1,1}(4,:)'"/1 -> dotprod4/1
  dotprod3/1 -> Mux/3
  "IW{1,1}(3,:)'"/1 -> dotprod3/1
  dotprod2/1 -> Mux/2
  "IW{1,1}(2,:)'"/1 -> dotprod2/1
  dotprod1/1 -> Mux/1
  "pd{1,1}"/1 -> dotprod100/2, dotprod99/2, dotprod98/2, dotprod97/2, dotprod96/2, dotprod95/2, dotprod94/2, dotprod93/2, dotprod92/2, dotprod91/2, dotprod90/2, dotprod89/2, dotprod88/2, dotprod87/2, dotprod86/2, dotprod85/2, dotprod84/2, dotprod83/2, dotprod82/2, dotprod81/2, dotprod80/2, dotprod79/2, dotprod78/2, dotprod77/2, dotprod76/2, dotprod75/2, dotprod74/2, dotprod73/2, dotprod72/2, dotprod71/2, dotprod70/2, dotprod69/2, dotprod68/2, dotprod67/2, dotprod66/2, dotprod65/2, dotprod64/2, dotprod63/2, dotprod62/2, dotprod61/2, dotprod60/2, dotprod59/2, dotprod58/2, dotprod57/2, dotprod56/2, dotprod55/2, dotprod54/2, dotprod53/2, dotprod52/2, dotprod51/2, dotprod50/2, dotprod49/2, dotprod48/2, dotprod47/2, dotprod46/2, dotprod45/2, dotprod44/2, dotprod43/2, dotprod42/2, dotprod41/2, dotprod40/2, dotprod39/2, dotprod38/2, dotprod37/2, dotprod36/2, dotprod35/2, dotprod34/2, dotprod33/2, dotprod32/2, dotprod31/2, dotprod30/2, dotprod29/2, dotprod28/2, dotprod27/2, dotprod26/2, dotprod25/2, dotprod24/2, dotprod23/2, dotprod22/2, dotprod21/2, dotprod20/2, dotprod19/2, dotprod18/2, dotprod17/2, dotprod16/2, dotprod15/2, dotprod14/2, dotprod13/2, dotprod12/2, dotprod11/2, dotprod10/2, dotprod9/2, dotprod8/2, dotprod7/2, dotprod6/2, dotprod5/2, dotprod4/2, dotprod3/2, dotprod2/2, dotprod1/2
  "IW{1,1}(1,:)'"/1 -> dotprod1/1
